simulink model "volo_agcdc_pipelined"  (R2012b)
settings: Solver=ode45  StartTime=0.0  StopTime=1000  RelTol=1e-3
PreLoadFcn:
  | volo_agcdc_init
InitFcn:
  | volo_agcdc_init
StartFcn:
  | volo_agcdc_init
values from neighbouring files (symbols this model uses):
  agc_idleState = 0    [volo_agcdc_init.m]
  agc_numAddrBits = agc_numOutputs + agc_numStateBits    [volo_agcdc_init.m]
  regDCRemoval_AvgLength = 64    [volo_agcdc_init.m]
  regSatDet_NumSamples = 16    [volo_agcdc_init.m]
undefined symbols (not defined in the file or in its folder): gcbh, xlBlockLoadCallback, xlGetNormalizedPeriod
libraries: xbsIndex_r4 x681, xbsEDKLib_r4 x1
(part 4 of 7)

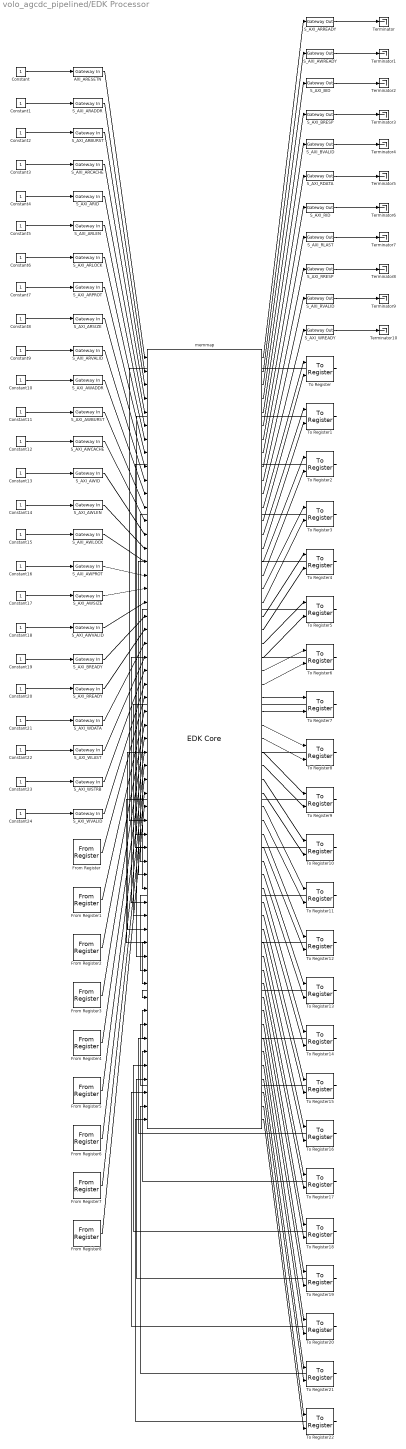
== system volo_agcdc_pipelined/EDK Processor ==
  AXI_ARESETN : xbsIndex_r4/Gateway In  gui_display_data_type=Fixed-point  arith_type=Boolean  n_bits=16  bin_pt=14  preci_type=Single  exp_width=8  frac_width=24  quantization="Round  (unbiased: +/- Inf)"  overflow=Saturate  period=xlGetNormalizedPeriod()  dbl_ovrd=off  timing_constraint=None  locs_specified=off  LOCs={}  UseAsADC=off  ADCChannel='1'  inherit_from_input=off  hdl_port=on  block_type=gatewayin
  Constant{,1..24} (25 alike) : Constant
  From Register : xbsIndex_r4/From Register  shared_memory_name='regSatDet_SaturationDetected'  init=0  period=xlGetNormalizedPeriod()  ownership=Owned and initialized elsewhere  gui_display_data_type=Fixed-point  arith_type=Unsigned  n_bits=1  bin_pt=0  preci_type=Single  dbl_ovrd=off  block_type=fromreg
      settings: AttributesFormatString=<< %<shared_memory_name> >>  infoedit="Register block that reads data to a shared memory register.  Delay of one sample period."
  From Register1 : xbsIndex_r4/From Register  shared_memory_name='regWSD_RXGAIN_READ'  init=0  period=xlGetNormalizedPeriod()  ownership=Owned and initialized elsewhere  gui_display_data_type=Fixed-point  arith_type="Signed  (2's comp)"  n_bits=9  bin_pt=0  preci_type=Single  dbl_ovrd=off  block_type=fromreg
      settings: AttributesFormatString=<< %<shared_memory_name> >>  infoedit="Register block that reads data to a shared memory register.  Delay of one sample period."
  From Register2 : xbsIndex_r4/From Register  shared_memory_name='regWSD_RSSI'  init=0  period=xlGetNormalizedPeriod()  ownership=Owned and initialized elsewhere  gui_display_data_type=Fixed-point  arith_type="Signed  (2's comp)"  n_bits=10  bin_pt=0  preci_type=Single  dbl_ovrd=off  block_type=fromreg
      settings: AttributesFormatString=<< %<shared_memory_name> >>  infoedit="Register block that reads data to a shared memory register.  Delay of one sample period."
  From Register3 : xbsIndex_r4/From Register  shared_memory_name='regWSD_meanPower'  init=0  period=xlGetNormalizedPeriod()  ownership=Owned and initialized elsewhere  gui_display_data_type=Fixed-point  arith_type="Signed  (2's comp)"  n_bits=9  bin_pt=0  preci_type=Single  dbl_ovrd=off  block_type=fromreg
      settings: AttributesFormatString=<< %<shared_memory_name> >>  infoedit="Register block that reads data to a shared memory register.  Delay of one sample period."
  From Register4 : xbsIndex_r4/From Register  shared_memory_name='regWSD_MeanDC_Q'  init=0  period=xlGetNormalizedPeriod()  ownership=Owned and initialized elsewhere  gui_display_data_type=Fixed-point  arith_type="Signed  (2's comp)"  n_bits=12  bin_pt=11  preci_type=Single  dbl_ovrd=off  block_type=fromreg
      settings: AttributesFormatString=<< %<shared_memory_name> >>  infoedit="Register block that reads data to a shared memory register.  Delay of one sample period."
  From Register5 : xbsIndex_r4/From Register  shared_memory_name='regWSD_MeanDC_I'  init=0  period=xlGetNormalizedPeriod()  ownership=Owned and initialized elsewhere  gui_display_data_type=Fixed-point  arith_type="Signed  (2's comp)"  n_bits=12  bin_pt=11  preci_type=Single  dbl_ovrd=off  block_type=fromreg
      settings: AttributesFormatString=<< %<shared_memory_name> >>  infoedit="Register block that reads data to a shared memory register.  Delay of one sample period."
  From Register6 : xbsIndex_r4/From Register  shared_memory_name='regWSD_RxLNAGain'  init=0  period=xlGetNormalizedPeriod()  ownership=Owned and initialized elsewhere  gui_display_data_type=Fixed-point  arith_type=Unsigned  n_bits=8  bin_pt=0  preci_type=Single  dbl_ovrd=off  block_type=fromreg
      settings: AttributesFormatString=<< %<shared_memory_name> >>  infoedit="Register block that reads data to a shared memory register.  Delay of one sample period."
  From Register7 : xbsIndex_r4/From Register  shared_memory_name='regWSD_RxVGA1Gain'  init=0  period=xlGetNormalizedPeriod()  ownership=Owned and initialized elsewhere  gui_display_data_type=Fixed-point  arith_type=Unsigned  n_bits=8  bin_pt=0  preci_type=Single  dbl_ovrd=off  block_type=fromreg
      settings: AttributesFormatString=<< %<shared_memory_name> >>  infoedit="Register block that reads data to a shared memory register.  Delay of one sample period."
  From Register8 : xbsIndex_r4/From Register  shared_memory_name='regWSD_RxVGA2Gain'  init=0  period=xlGetNormalizedPeriod()  ownership=Owned and initialized elsewhere  gui_display_data_type=Fixed-point  arith_type=Unsigned  n_bits=8  bin_pt=0  preci_type=Single  dbl_ovrd=off  block_type=fromreg
      settings: AttributesFormatString=<< %<shared_memory_name> >>  infoedit="Register block that reads data to a shared memory register.  Delay of one sample period."
  S_AXI_ARADDR : xbsIndex_r4/Gateway In  gui_display_data_type=Fixed-point  arith_type=Unsigned  n_bits=32  bin_pt=0  preci_type=Single  exp_width=8  frac_width=24  quantization="Round  (unbiased: +/- Inf)"  overflow=Saturate  period=xlGetNormalizedPeriod()  dbl_ovrd=off  timing_constraint=None  locs_specified=off  LOCs={}  UseAsADC=off  ADCChannel='1'  inherit_from_input=off  hdl_port=on  block_type=gatewayin
  S_AXI_ARBURST : xbsIndex_r4/Gateway In  gui_display_data_type=Fixed-point  arith_type=Unsigned  n_bits=2  bin_pt=0  preci_type=Single  exp_width=8  frac_width=24  quantization="Round  (unbiased: +/- Inf)"  overflow=Saturate  period=xlGetNormalizedPeriod()  dbl_ovrd=off  timing_constraint=None  locs_specified=off  LOCs={}  UseAsADC=off  ADCChannel='1'  inherit_from_input=off  hdl_port=on  block_type=gatewayin
  S_AXI_ARCACHE : xbsIndex_r4/Gateway In  gui_display_data_type=Fixed-point  arith_type=Unsigned  n_bits=4  bin_pt=0  preci_type=Single  exp_width=8  frac_width=24  quantization="Round  (unbiased: +/- Inf)"  overflow=Saturate  period=xlGetNormalizedPeriod()  dbl_ovrd=off  timing_constraint=None  locs_specified=off  LOCs={}  UseAsADC=off  ADCChannel='1'  inherit_from_input=off  hdl_port=on  block_type=gatewayin
  S_AXI_ARID : xbsIndex_r4/Gateway In  gui_display_data_type=Fixed-point  arith_type=Unsigned  n_bits=8  bin_pt=0  preci_type=Single  exp_width=8  frac_width=24  quantization="Round  (unbiased: +/- Inf)"  overflow=Saturate  period=xlGetNormalizedPeriod()  dbl_ovrd=off  timing_constraint=None  locs_specified=off  LOCs={}  UseAsADC=off  ADCChannel='1'  inherit_from_input=off  hdl_port=on  block_type=gatewayin
  S_AXI_ARLEN : xbsIndex_r4/Gateway In  gui_display_data_type=Fixed-point  arith_type=Unsigned  n_bits=8  bin_pt=0  preci_type=Single  exp_width=8  frac_width=24  quantization="Round  (unbiased: +/- Inf)"  overflow=Saturate  period=xlGetNormalizedPeriod()  dbl_ovrd=off  timing_constraint=None  locs_specified=off  LOCs={}  UseAsADC=off  ADCChannel='1'  inherit_from_input=off  hdl_port=on  block_type=gatewayin
  S_AXI_ARLOCK : xbsIndex_r4/Gateway In  gui_display_data_type=Fixed-point  arith_type=Unsigned  n_bits=2  bin_pt=0  preci_type=Single  exp_width=8  frac_width=24  quantization="Round  (unbiased: +/- Inf)"  overflow=Saturate  period=xlGetNormalizedPeriod()  dbl_ovrd=off  timing_constraint=None  locs_specified=off  LOCs={}  UseAsADC=off  ADCChannel='1'  inherit_from_input=off  hdl_port=on  block_type=gatewayin
  S_AXI_ARPROT : xbsIndex_r4/Gateway In  gui_display_data_type=Fixed-point  arith_type=Unsigned  n_bits=3  bin_pt=0  preci_type=Single  exp_width=8  frac_width=24  quantization="Round  (unbiased: +/- Inf)"  overflow=Saturate  period=xlGetNormalizedPeriod()  dbl_ovrd=off  timing_constraint=None  locs_specified=off  LOCs={}  UseAsADC=off  ADCChannel='1'  inherit_from_input=off  hdl_port=on  block_type=gatewayin
  S_AXI_ARREADY : xbsIndex_r4/Gateway Out  inherit_from_input=off  hdl_port=on  timing_constraint=None  locs_specified=off  LOCs={}  UseAsDAC=off  DACChannel='1'  block_type=gatewayout
  S_AXI_ARSIZE : xbsIndex_r4/Gateway In  gui_display_data_type=Fixed-point  arith_type=Unsigned  n_bits=3  bin_pt=0  preci_type=Single  exp_width=8  frac_width=24  quantization="Round  (unbiased: +/- Inf)"  overflow=Saturate  period=xlGetNormalizedPeriod()  dbl_ovrd=off  timing_constraint=None  locs_specified=off  LOCs={}  UseAsADC=off  ADCChannel='1'  inherit_from_input=off  hdl_port=on  block_type=gatewayin
  S_AXI_ARVALID : xbsIndex_r4/Gateway In  gui_display_data_type=Fixed-point  arith_type=Boolean  n_bits=16  bin_pt=14  preci_type=Single  exp_width=8  frac_width=24  quantization="Round  (unbiased: +/- Inf)"  overflow=Saturate  period=xlGetNormalizedPeriod()  dbl_ovrd=off  timing_constraint=None  locs_specified=off  LOCs={}  UseAsADC=off  ADCChannel='1'  inherit_from_input=off  hdl_port=on  block_type=gatewayin
  S_AXI_AWADDR : xbsIndex_r4/Gateway In  gui_display_data_type=Fixed-point  arith_type=Unsigned  n_bits=32  bin_pt=0  preci_type=Single  exp_width=8  frac_width=24  quantization="Round  (unbiased: +/- Inf)"  overflow=Saturate  period=xlGetNormalizedPeriod()  dbl_ovrd=off  timing_constraint=None  locs_specified=off  LOCs={}  UseAsADC=off  ADCChannel='1'  inherit_from_input=off  hdl_port=on  block_type=gatewayin
  S_AXI_AWBURST : xbsIndex_r4/Gateway In  gui_display_data_type=Fixed-point  arith_type=Unsigned  n_bits=2  bin_pt=0  preci_type=Single  exp_width=8  frac_width=24  quantization="Round  (unbiased: +/- Inf)"  overflow=Saturate  period=xlGetNormalizedPeriod()  dbl_ovrd=off  timing_constraint=None  locs_specified=off  LOCs={}  UseAsADC=off  ADCChannel='1'  inherit_from_input=off  hdl_port=on  block_type=gatewayin
  S_AXI_AWCACHE : xbsIndex_r4/Gateway In  gui_display_data_type=Fixed-point  arith_type=Unsigned  n_bits=4  bin_pt=0  preci_type=Single  exp_width=8  frac_width=24  quantization="Round  (unbiased: +/- Inf)"  overflow=Saturate  period=xlGetNormalizedPeriod()  dbl_ovrd=off  timing_constraint=None  locs_specified=off  LOCs={}  UseAsADC=off  ADCChannel='1'  inherit_from_input=off  hdl_port=on  block_type=gatewayin
  S_AXI_AWID : xbsIndex_r4/Gateway In  gui_display_data_type=Fixed-point  arith_type=Unsigned  n_bits=8  bin_pt=0  preci_type=Single  exp_width=8  frac_width=24  quantization="Round  (unbiased: +/- Inf)"  overflow=Saturate  period=xlGetNormalizedPeriod()  dbl_ovrd=off  timing_constraint=None  locs_specified=off  LOCs={}  UseAsADC=off  ADCChannel='1'  inherit_from_input=off  hdl_port=on  block_type=gatewayin
  S_AXI_AWLEN : xbsIndex_r4/Gateway In  gui_display_data_type=Fixed-point  arith_type=Unsigned  n_bits=8  bin_pt=0  preci_type=Single  exp_width=8  frac_width=24  quantization="Round  (unbiased: +/- Inf)"  overflow=Saturate  period=xlGetNormalizedPeriod()  dbl_ovrd=off  timing_constraint=None  locs_specified=off  LOCs={}  UseAsADC=off  ADCChannel='1'  inherit_from_input=off  hdl_port=on  block_type=gatewayin
  S_AXI_AWLOCK : xbsIndex_r4/Gateway In  gui_display_data_type=Fixed-point  arith_type=Unsigned  n_bits=2  bin_pt=0  preci_type=Single  exp_width=8  frac_width=24  quantization="Round  (unbiased: +/- Inf)"  overflow=Saturate  period=xlGetNormalizedPeriod()  dbl_ovrd=off  timing_constraint=None  locs_specified=off  LOCs={}  UseAsADC=off  ADCChannel='1'  inherit_from_input=off  hdl_port=on  block_type=gatewayin
  S_AXI_AWPROT : xbsIndex_r4/Gateway In  gui_display_data_type=Fixed-point  arith_type=Unsigned  n_bits=3  bin_pt=0  preci_type=Single  exp_width=8  frac_width=24  quantization="Round  (unbiased: +/- Inf)"  overflow=Saturate  period=xlGetNormalizedPeriod()  dbl_ovrd=off  timing_constraint=None  locs_specified=off  LOCs={}  UseAsADC=off  ADCChannel='1'  inherit_from_input=off  hdl_port=on  block_type=gatewayin
  S_AXI_AWREADY : xbsIndex_r4/Gateway Out  inherit_from_input=off  hdl_port=on  timing_constraint=None  locs_specified=off  LOCs={}  UseAsDAC=off  DACChannel='1'  block_type=gatewayout
  S_AXI_AWSIZE : xbsIndex_r4/Gateway In  gui_display_data_type=Fixed-point  arith_type=Unsigned  n_bits=3  bin_pt=0  preci_type=Single  exp_width=8  frac_width=24  quantization="Round  (unbiased: +/- Inf)"  overflow=Saturate  period=xlGetNormalizedPeriod()  dbl_ovrd=off  timing_constraint=None  locs_specified=off  LOCs={}  UseAsADC=off  ADCChannel='1'  inherit_from_input=off  hdl_port=on  block_type=gatewayin
  S_AXI_AWVALID : xbsIndex_r4/Gateway In  gui_display_data_type=Fixed-point  arith_type=Boolean  n_bits=16  bin_pt=14  preci_type=Single  exp_width=8  frac_width=24  quantization="Round  (unbiased: +/- Inf)"  overflow=Saturate  period=xlGetNormalizedPeriod()  dbl_ovrd=off  timing_constraint=None  locs_specified=off  LOCs={}  UseAsADC=off  ADCChannel='1'  inherit_from_input=off  hdl_port=on  block_type=gatewayin
  S_AXI_BID : xbsIndex_r4/Gateway Out  inherit_from_input=off  hdl_port=on  timing_constraint=None  locs_specified=off  LOCs={}  UseAsDAC=off  DACChannel='1'  block_type=gatewayout
  S_AXI_BREADY : xbsIndex_r4/Gateway In  gui_display_data_type=Fixed-point  arith_type=Boolean  n_bits=16  bin_pt=14  preci_type=Single  exp_width=8  frac_width=24  quantization="Round  (unbiased: +/- Inf)"  overflow=Saturate  period=xlGetNormalizedPeriod()  dbl_ovrd=off  timing_constraint=None  locs_specified=off  LOCs={}  UseAsADC=off  ADCChannel='1'  inherit_from_input=off  hdl_port=on  block_type=gatewayin
  S_AXI_BRESP : xbsIndex_r4/Gateway Out  inherit_from_input=off  hdl_port=on  timing_constraint=None  locs_specified=off  LOCs={}  UseAsDAC=off  DACChannel='1'  block_type=gatewayout
  S_AXI_BVALID : xbsIndex_r4/Gateway Out  inherit_from_input=off  hdl_port=on  timing_constraint=None  locs_specified=off  LOCs={}  UseAsDAC=off  DACChannel='1'  block_type=gatewayout
  S_AXI_RDATA : xbsIndex_r4/Gateway Out  inherit_from_input=off  hdl_port=on  timing_constraint=None  locs_specified=off  LOCs={}  UseAsDAC=off  DACChannel='1'  block_type=gatewayout
  S_AXI_RID : xbsIndex_r4/Gateway Out  inherit_from_input=off  hdl_port=on  timing_constraint=None  locs_specified=off  LOCs={}  UseAsDAC=off  DACChannel='1'  block_type=gatewayout
  S_AXI_RLAST : xbsIndex_r4/Gateway Out  inherit_from_input=off  hdl_port=on  timing_constraint=None  locs_specified=off  LOCs={}  UseAsDAC=off  DACChannel='1'  block_type=gatewayout
  S_AXI_RREADY : xbsIndex_r4/Gateway In  gui_display_data_type=Fixed-point  arith_type=Boolean  n_bits=16  bin_pt=14  preci_type=Single  exp_width=8  frac_width=24  quantization="Round  (unbiased: +/- Inf)"  overflow=Saturate  period=xlGetNormalizedPeriod()  dbl_ovrd=off  timing_constraint=None  locs_specified=off  LOCs={}  UseAsADC=off  ADCChannel='1'  inherit_from_input=off  hdl_port=on  block_type=gatewayin
  S_AXI_RRESP : xbsIndex_r4/Gateway Out  inherit_from_input=off  hdl_port=on  timing_constraint=None  locs_specified=off  LOCs={}  UseAsDAC=off  DACChannel='1'  block_type=gatewayout
  S_AXI_RVALID : xbsIndex_r4/Gateway Out  inherit_from_input=off  hdl_port=on  timing_constraint=None  locs_specified=off  LOCs={}  UseAsDAC=off  DACChannel='1'  block_type=gatewayout
  S_AXI_WDATA : xbsIndex_r4/Gateway In  gui_display_data_type=Fixed-point  arith_type=Unsigned  n_bits=32  bin_pt=0  preci_type=Single  exp_width=8  frac_width=24  quantization="Round  (unbiased: +/- Inf)"  overflow=Saturate  period=xlGetNormalizedPeriod()  dbl_ovrd=off  timing_constraint=None  locs_specified=off  LOCs={}  UseAsADC=off  ADCChannel='1'  inherit_from_input=off  hdl_port=on  block_type=gatewayin
  S_AXI_WLAST : xbsIndex_r4/Gateway In  gui_display_data_type=Fixed-point  arith_type=Boolean  n_bits=16  bin_pt=14  preci_type=Single  exp_width=8  frac_width=24  quantization="Round  (unbiased: +/- Inf)"  overflow=Saturate  period=xlGetNormalizedPeriod()  dbl_ovrd=off  timing_constraint=None  locs_specified=off  LOCs={}  UseAsADC=off  ADCChannel='1'  inherit_from_input=off  hdl_port=on  block_type=gatewayin
  S_AXI_WREADY : xbsIndex_r4/Gateway Out  inherit_from_input=off  hdl_port=on  timing_constraint=None  locs_specified=off  LOCs={}  UseAsDAC=off  DACChannel='1'  block_type=gatewayout
  S_AXI_WSTRB : xbsIndex_r4/Gateway In  gui_display_data_type=Fixed-point  arith_type=Unsigned  n_bits=4  bin_pt=0  preci_type=Single  exp_width=8  frac_width=24  quantization="Round  (unbiased: +/- Inf)"  overflow=Saturate  period=xlGetNormalizedPeriod()  dbl_ovrd=off  timing_constraint=None  locs_specified=off  LOCs={}  UseAsADC=off  ADCChannel='1'  inherit_from_input=off  hdl_port=on  block_type=gatewayin
  S_AXI_WVALID : xbsIndex_r4/Gateway In  gui_display_data_type=Fixed-point  arith_type=Boolean  n_bits=16  bin_pt=14  preci_type=Single  exp_width=8  frac_width=24  quantization="Round  (unbiased: +/- Inf)"  overflow=Saturate  period=xlGetNormalizedPeriod()  dbl_ovrd=off  timing_constraint=None  locs_specified=off  LOCs={}  UseAsADC=off  ADCChannel='1'  inherit_from_input=off  hdl_port=on  block_type=gatewayin
  Terminator{,1..10} (11 alike) : Terminator
  To Register : xbsIndex_r4/To Register  shared_memory_name='regAGC_DefaultGainSettings'  init=0  ownership=Owned and initialized elsewhere  explicit_data_type=on  gui_display_data_type=Fixed-point  arith_type=Unsigned  n_bits=32  bin_pt=0  preci_type=Single  dbl_ovrd=off  block_type=toreg
      settings: AttributesFormatString=<< %<shared_memory_name> >>  infoedit="Register block that writes data to a shared memory register.  Delay of one sample period."
  To Register1 : xbsIndex_r4/To Register  shared_memory_name='regSPICtrl_SPIWriteDelay'  init=0  ownership=Owned and initialized elsewhere  explicit_data_type=on  gui_display_data_type=Fixed-point  arith_type=Unsigned  n_bits=8  bin_pt=0  preci_type=Single  dbl_ovrd=off  block_type=toreg
      settings: AttributesFormatString=<< %<shared_memory_name> >>  infoedit="Register block that writes data to a shared memory register.  Delay of one sample period."
  To Register10 : xbsIndex_r4/To Register  shared_memory_name='regAGC_WSDAGCCtrl'  init=0  ownership=Owned and initialized elsewhere  explicit_data_type=on  gui_display_data_type=Fixed-point  arith_type=Unsigned  n_bits=32  bin_pt=0  preci_type=Single  dbl_ovrd=off  block_type=toreg
      settings: AttributesFormatString=<< %<shared_memory_name> >>  infoedit="Register block that writes data to a shared memory register.  Delay of one sample period."
  To Register11 : xbsIndex_r4/To Register  shared_memory_name='regAGC_AutoCorr_RatioThresh'  init=0  ownership=Owned and initialized elsewhere  explicit_data_type=on  gui_display_data_type=Fixed-point  arith_type=Unsigned  n_bits=8  bin_pt=8  preci_type=Single  dbl_ovrd=off  block_type=toreg
      settings: AttributesFormatString=<< %<shared_memory_name> >>  infoedit="Register block that writes data to a shared memory register.  Delay of one sample period."
  To Register12 : xbsIndex_r4/To Register  shared_memory_name='regAGC_ManualRxVGA1_Gain'  init=0  ownership=Owned and initialized elsewhere  explicit_data_type=on  gui_display_data_type=Fixed-point  arith_type=Unsigned  n_bits=8  bin_pt=0  preci_type=Single  dbl_ovrd=off  block_type=toreg
      settings: AttributesFormatString=<< %<shared_memory_name> >>  infoedit="Register block that writes data to a shared memory register.  Delay of one sample period."
  To Register13 : xbsIndex_r4/To Register  shared_memory_name='regAGC_ManualRxLNA_Gain'  init=0  ownership=Owned and initialized elsewhere  explicit_data_type=on  gui_display_data_type=Fixed-point  arith_type=Unsigned  n_bits=8  bin_pt=0  preci_type=Single  dbl_ovrd=off  block_type=toreg
      settings: AttributesFormatString=<< %<shared_memory_name> >>  infoedit="Register block that writes data to a shared memory register.  Delay of one sample period."
  To Register14 : xbsIndex_r4/To Register  shared_memory_name='regAGC_ManualRxVGA2_Gain'  init=0  ownership=Owned and initialized elsewhere  explicit_data_type=on  gui_display_data_type=Fixed-point  arith_type=Unsigned  n_bits=8  bin_pt=0  preci_type=Single  dbl_ovrd=off  block_type=toreg
      settings: AttributesFormatString=<< %<shared_memory_name> >>  infoedit="Register block that writes data to a shared memory register.  Delay of one sample period."
  To Register15 : xbsIndex_r4/To Register  shared_memory_name='regAGC_AutoCorr_LagTime'  init=0  ownership=Owned and initialized elsewhere  explicit_data_type=on  gui_display_data_type=Fixed-point  arith_type=Unsigned  n_bits=12  bin_pt=0  preci_type=Single  dbl_ovrd=off  block_type=toreg
      settings: AttributesFormatString=<< %<shared_memory_name> >>  infoedit="Register block that writes data to a shared memory register.  Delay of one sample period."
  To Register16 : xbsIndex_r4/To Register  shared_memory_name='regAGC_pktDetPwr_absoluteThreshold_dBm'  init=0  ownership=Owned and initialized elsewhere  explicit_data_type=on  gui_display_data_type=Fixed-point  arith_type="Signed  (2's comp)"  n_bits=9  bin_pt=0  preci_type=Single  dbl_ovrd=off  block_type=toreg
      settings: AttributesFormatString=<< %<shared_memory_name> >>  infoedit="Register block that writes data to a shared memory register.  Delay of one sample period."
  To Register17 : xbsIndex_r4/To Register  shared_memory_name='regAGC_pktDetPwr_detectLag'  init=0  ownership=Owned and initialized elsewhere  explicit_data_type=on  gui_display_data_type=Fixed-point  arith_type=Unsigned  n_bits=6  bin_pt=0  preci_type=Single  dbl_ovrd=off  block_type=toreg
      settings: AttributesFormatString=<< %<shared_memory_name> >>  infoedit="Register block that writes data to a shared memory register.  Delay of one sample period."
  To Register18 : xbsIndex_r4/To Register  shared_memory_name='regAGC_NumFineGainSteps'  init=0  ownership=Owned and initialized elsewhere  explicit_data_type=on  gui_display_data_type=Fixed-point  arith_type=Unsigned  n_bits=4  bin_pt=0  preci_type=Single  dbl_ovrd=off  block_type=toreg
      settings: AttributesFormatString=<< %<shared_memory_name> >>  infoedit="Register block that writes data to a shared memory register.  Delay of one sample period."
  To Register19 : xbsIndex_r4/To Register  shared_memory_name='regAGC_WSD_CCAThreshold_dBm'  init=0  ownership=Owned and initialized elsewhere  explicit_data_type=on  gui_display_data_type=Fixed-point  arith_type=Unsigned  n_bits=10  bin_pt=0  preci_type=Single  dbl_ovrd=off  block_type=toreg
      settings: AttributesFormatString=<< %<shared_memory_name> >>  infoedit="Register block that writes data to a shared memory register.  Delay of one sample period."
  To Register2 : xbsIndex_r4/To Register  shared_memory_name='regPwrMeas_AvgLength'  init=0  ownership=Owned and initialized elsewhere  explicit_data_type=on  gui_display_data_type=Fixed-point  arith_type=Unsigned  n_bits=7  bin_pt=0  preci_type=Single  dbl_ovrd=off  block_type=toreg
      settings: AttributesFormatString=<< %<shared_memory_name> >>  infoedit="Register block that writes data to a shared memory register.  Delay of one sample period."
  To Register20 : xbsIndex_r4/To Register  shared_memory_name='regAGC_LongCorr_Threshold'  init=0  ownership=Owned and initialized elsewhere  explicit_data_type=on  gui_display_data_type=Fixed-point  arith_type=Unsigned  n_bits=32  bin_pt=0  preci_type=Single  dbl_ovrd=off  block_type=toreg
      settings: AttributesFormatString=<< %<shared_memory_name> >>  infoedit="Register block that writes data to a shared memory register.  Delay of one sample period."
  To Register21 : xbsIndex_r4/To Register  shared_memory_name='regAGC_pktDetPwr_deltaThreshold_dBm'  init=0  ownership=Owned and initialized elsewhere  explicit_data_type=on  gui_display_data_type=Fixed-point  arith_type="Signed  (2's comp)"  n_bits=9  bin_pt=0  preci_type=Single  dbl_ovrd=off  block_type=toreg
      settings: AttributesFormatString=<< %<shared_memory_name> >>  infoedit="Register block that writes data to a shared memory register.  Delay of one sample period."
  To Register22 : xbsIndex_r4/To Register  shared_memory_name='regAGC_SPITIMINGFUDGE'  init=0  ownership=Owned and initialized elsewhere  explicit_data_type=on  gui_display_data_type=Fixed-point  arith_type=Unsigned  n_bits=12  bin_pt=0  preci_type=Single  dbl_ovrd=off  block_type=toreg
      settings: AttributesFormatString=<< %<shared_memory_name> >>  infoedit="Register block that writes data to a shared memory register.  Delay of one sample period."
  To Register3 : xbsIndex_r4/To Register  shared_memory_name='regSatDet_SaturationMaxCount'  init=0  ownership=Owned and initialized elsewhere  explicit_data_type=on  gui_display_data_type=Fixed-point  arith_type=Unsigned  n_bits=6  bin_pt=0  preci_type=Single  dbl_ovrd=off  block_type=toreg
      settings: AttributesFormatString=<< %<shared_memory_name> >>  infoedit="Register block that writes data to a shared memory register.  Delay of one sample period."
  To Register4 : xbsIndex_r4/To Register  shared_memory_name='regSatDet_NumSamples'  init=0  ownership=Owned and initialized elsewhere  explicit_data_type=on  gui_display_data_type=Fixed-point  arith_type=Unsigned  n_bits=5  bin_pt=0  preci_type=Single  dbl_ovrd=off  block_type=toreg
      settings: AttributesFormatString=<< %<shared_memory_name> >>  infoedit="Register block that writes data to a shared memory register.  Delay of one sample period."
  To Register5 : xbsIndex_r4/To Register  shared_memory_name='regSatDet_SaturationThreshold'  init=0  ownership=Owned and initialized elsewhere  explicit_data_type=on  gui_display_data_type=Fixed-point  arith_type="Signed  (2's comp)"  n_bits=14  bin_pt=13  preci_type=Single  dbl_ovrd=off  block_type=toreg
      settings: AttributesFormatString=<< %<shared_memory_name> >>  infoedit="Register block that writes data to a shared memory register.  Delay of one sample period."
  To Register6 : xbsIndex_r4/To Register  shared_memory_name='regAGC_ExtPktDet_DelayCount'  init=0  ownership=Owned and initialized elsewhere  explicit_data_type=on  gui_display_data_type=Fixed-point  arith_type=Unsigned  n_bits=32  bin_pt=0  preci_type=Single  dbl_ovrd=off  block_type=toreg
      settings: AttributesFormatString=<< %<shared_memory_name> >>  infoedit="Register block that writes data to a shared memory register.  Delay of one sample period."
  To Register7 : xbsIndex_r4/To Register  shared_memory_name='regAGC_targetRxInputPwr'  init=0  ownership=Owned and initialized elsewhere  explicit_data_type=on  gui_display_data_type=Fixed-point  arith_type="Signed  (2's comp)"  n_bits=9  bin_pt=0  preci_type=Single  dbl_ovrd=off  block_type=toreg
      settings: AttributesFormatString=<< %<shared_memory_name> >>  infoedit="Register block that writes data to a shared memory register.  Delay of one sample period."
  To Register8 : xbsIndex_r4/To Register  shared_memory_name='regAGC_AutoCorr_MinPower'  init=0  ownership=Owned and initialized elsewhere  explicit_data_type=on  gui_display_data_type=Fixed-point  arith_type=Unsigned  n_bits=16  bin_pt=8  preci_type=Single  dbl_ovrd=off  block_type=toreg
      settings: AttributesFormatString=<< %<shared_memory_name> >>  infoedit="Register block that writes data to a shared memory register.  Delay of one sample period."
  To Register9 : xbsIndex_r4/To Register  shared_memory_name='regAGC_AutoCorr_MinPktDuration'  init=0  ownership=Owned and initialized elsewhere  explicit_data_type=on  gui_display_data_type=Fixed-point  arith_type=Unsigned  n_bits=6  bin_pt=0  preci_type=Single  dbl_ovrd=off  block_type=toreg
      settings: AttributesFormatString=<< %<shared_memory_name> >>  infoedit="Register block that writes data to a shared memory register.  Delay of one sample period."
  memmap : xbsEDKLib_r4/EDK Core  sim_method=Inactive  xmp=xmp  blockname=blockname  dual_clock=dual_clock  procinfo=procinfo  bus_type=bus_type  memxtable=memxtable  memmap_hdlcontent=|  config={'inports'=>[{'arith_type'=>2.00000000000000000,'bin_pt'=>0.00000000000000000,'name'=>'AXI_ARESETN','width'=>0},{'arith_type'=>2.00000000000000000,'bin_pt'=>0.00000000000000000,'name'=>'S_AXI_ARADDR','width'=>32},{'arith_type'=>2.00000000000000000,'bin_pt'=>0.00000000000000000,'name'=>'S_AXI_ARBURST','width'=>2},{'arith_type'=>2.00000000000000000,'bin_pt'=>0.00000000000000000,'name'=>'S_AXI_ARCACHE','width'=>4},{'arith_type'=>2.00000000000000000,'bin_pt'=>0.00000000000000000,'name'=>'S_AXI_ARID','width'=>8},{'arith_type'=>2.00000000000000000,'bin_pt'=>0.00000000000000000,'name'=>'S_AXI_ARLEN','width'=>8},{'arith_type'=>2.00000000000000000,'bin_pt'=>0.00000000000000000,'name'=>'S_AXI_ARLOCK','width'=>2},{'arith_type'=>2.00000000000000000,'bin_pt'=>0.00000000000000000,'name'=>'S_AXI_ARPROT','width'=>3},{'arith_type'=>2.00000000000000000,'bin_pt'=>0.00000000000000000,'name'=>'S_AXI_ARSIZE','width'=>3},{'arith_type'=>2.00000000000000000,'bin_pt'=>0.00000000000000000,'name'=>'S_AXI_ARVALID','width'=>0},{'arith_type'=>2.00000000000000000,'bin_pt'=>0.00000000000000000,'name'=>'S_AXI_AWADDR','width'=>32},{'arith_type'=>2.00000000000000000,'bin_pt'=>0.00000000000000000,'name'=>'S_AXI_AWBURST','width'=>2},{'arith_type'=>2.00000000000000000,'bin_pt'=>0.00000000000000000,'name'=>'S_AXI_AWCACHE','width'=>4},{'arith_type'=>2.00000000000000000,'bin_pt'=>0.00000000000000000,'name'=>'S_AXI_AWID','width'=>8},{'arith_type'=>2.00000000000000000,'bin_pt'=>0.00000000000000000,'name'=>'S_AXI_AWLEN','width'=>8},{'arith_type'=>2.00000000000000000,'bin_pt'=>0.00000000000000000,'name'=>'S_AXI_AWLOCK','width'=>2},{'arith_type'=>2.00000000000000000,'bin_pt'=>0.00000000000000000,'name'=>'S_AXI_AWPROT','width'=>3},{'arith_type'=>2.00000000000000000,'bin_pt'=>0.00000000000000000,'name'=>'S_AXI_AWSIZE','width'=>3},{'arith_type'=>2.00000000000000000,'bin_pt'=>0.00000000000000000,'name'=>'S_AXI_AWVALID','width'=>0},{'arith_type'=>2.00000000000000000,'bin_pt'=>0.00000000000000000,'name'=>'S_AXI_BREADY','width'=>0},{'arith_type'=>2.00000000000000000,'bin_pt'=>0.00000000000000000,'name'=>'S_AXI_RREADY','width'=>0},{'arith_type'=>2.00000000000000000,'bin_pt'=>0.00000000000000000,'name'=>'S_AXI_WDATA','width'=>32},{'arith_type'=>2.00000000000000000,'bin_pt'=>0.00000000000000000,'name'=>'S_AXI_WLAST','width'=>0},{'arith_type'=>2.00000000000000000,'bin_pt'=>0.00000000000000000,'name'=>'S_AXI_WSTRB','width'=>4},{'arith_type'=>2.00000000000000000,'bin_pt'=>0.00000000000000000,'name'=>'S_AXI_WVALID','width'=>0},{'arith_type'=>2,'bin_pt'=>0,'name'=>'sm_regSatDet_SaturationDetected_dout','width'=>1},{'arith_type'=>1,'bin_pt'=>0,'name'=>'sm_regWSD_RXGAIN_READ_dout','width'=>9},{'arith_type'=>1,'bin_pt'=>0,'name'=>'sm_regWSD_RSSI_dout','width'=>10},{'arith_type'=>1,'bin_pt'=>0,'name'=>'sm_regWSD_meanPower_dout','width'=>9},{'arith_type'=>1,'bin_pt'=>11,'name'=>'sm_regWSD_MeanDC_Q_dout','width'=>12},{'arith_type'=>1,'bin_pt'=>11,'name'=>'sm_regWSD_MeanDC_I_dout','width'=>12},{'arith_type'=>2,'bin_pt'=>0,'name'=>'sm_regWSD_RxLNAGain_dout','width'=>8},{'arith_type'=>2,'bin_pt'=>0,'name'=>'sm_regWSD_RxVGA1Gain_dout','width'=>8},{'arith_type'=>2,'bin_pt'=>0,'name'=>'sm_regWSD_RxVGA2Gain_dout','width'=>8},{'arith_type'=>2,'bin_pt'=>0,'name'=>'sm_regAGC_DefaultGainSettings_dout','width'=>32},{'arith_type'=>2,'bin_pt'=>0,'name'=>'sm_regSPICtrl_SPIWriteDelay_dout','width'=>8},{'arith_type'=>2,'bin_pt'=>0,'name'=>'sm_regPwrMeas_AvgLength_dout','width'=>7},{'arith_type'=>2,'bin_pt'=>0,'name'=>'sm_regSatDet_SaturationMaxCount_dout','width'=>6},{'arith_type'=>2,'bin_pt'=>0,'name'=>'sm_regSatDet_NumSamples_dout','width'=>5},{'arith_type'=>1,'bin_pt'=>13,'name'=>'sm_regSatDet_SaturationThreshold_dout','width'=>14},{'arith_type'=>2,'bin_pt'=>0,'name'=>'sm_regAGC_ExtPktDet_DelayCount_dout','width'=>32},{'arith_type'=>1,'bin_pt'=>0,'name'=>'sm_regAGC_targetRxInputPwr_dout','width'=>9},{'arith_type'=>2,'bin_pt'=>8,'name'=>'sm_regAGC_AutoCorr_MinPower_dout','width'=>16},{'arith_type'=>2,'bin_pt'=>0,'name'=>'sm_regAGC_AutoCorr_MinPktDuration_dout','width'=>6},{'arith_type'=>2,'bin_pt'=>0,'name'=>'sm_regAGC_WSDAGCCtrl_dout','width'=>32},{'arith_type'=>2,'bin_pt'=>8,'name'=>'sm_regAGC_AutoCorr_RatioThresh_dout','width'=>8},{'arith_type'=>2,'bin_pt'=>0,'name'=>'sm_regAGC_ManualRxVGA1_Gain_dout','width'=>8},{'arith_type'=>2,'bin_pt'=>0,'name'=>'sm_regAGC_ManualRxLNA_Gain_dout','width'=>8},{'arith_type'=>2,'bin_pt'=>0,'name'=>'sm_regAGC_ManualRxVGA2_Gain_dout','width'=>8},{'arith_type'=>2,'bin_pt'=>0,'name'=>'sm_regAGC_AutoCorr_LagTime_dout','width'=>12},{'arith_type'=>1,'bin_pt'=>0,'name'=>'sm_regAGC_pktDetPwr_absoluteThreshold_dBm_dout','width'=>9},{'arith_type'=>2,'bin_pt'=>0,'name'=>'sm_regAGC_pktDetPwr_detectLag_dout','width'=>6},{'arith_type'=>2,'bin_pt'=>0,'name'=>'sm_regAGC_NumFineGainSteps_dout','width'=>4},{'arith_type'=>2,'bin_pt'=>0,'name'=>'sm_regAGC_WSD_CCAThreshold_dBm_dout','width'=>10},{'arith_type'=>2,'bin_pt'=>0,'name'=>'sm_regAGC_LongCorr_Threshold_dout','width'=>32},{'arith_type'=>1,'bin_pt'=>0,'name'=>'sm_regAGC_pktDetPwr_deltaThreshold_dBm_dout','width'=>9},{'arith_type'=>2,'bin_pt'=>0,'name'=>'sm_regAGC_SPITIMINGFUDGE_dout','width'=>12}],'outports'=>[{'arith_type'=>2.00000000000000000,'bin_pt'=>0.00000000000000000,'name'=>'S_AXI_ARREADY','width'=>0},{'arith_type'=>2.00000000000000000,'bin_pt'=>0.00000000000000000,'name'=>'S_AXI_AWREADY','width'=>0},{'arith_type'=>2.00000000000000000,'bin_pt'=>0.00000000000000000,'name'=>'S_AXI_BID','width'=>8},{'arith_type'=>2.00000000000000000,'bin_pt'=>0.00000000000000000,'name'=>'S_AXI_BRESP','width'=>2},{'arith_type'=>2.00000000000000000,'bin_pt'=>0.00000000000000000,'name'=>'S_AXI_BVALID','width'=>0},{'arith_type'=>2.00000000000000000,'bin_pt'=>0.00000000000000000,'name'=>'S_AXI_RDATA','width'=>32},{'arith_type'=>2.00000000000000000,'bin_pt'=>0.00000000000000000,'name'=>'S_AXI_RID','width'=>8},{'arith_type'=>2.00000000000000000,'bin_pt'=>0.00000000000000000,'name'=>'S_AXI_RLAST','width'=>0},{'arith_type'=>2.00000000000000000,'bin_pt'=>0.00000000000000000,'name'=>'S_AXI_RRESP','width'=>2},{'arith_type'=>2.00000000000000000,'bin_pt'=>0.00000000000000000,'name'=>'S_AXI_RVALID','width'=>0},{'arith_type'=>2.00000000000000000,'bin_pt'=>0.00000000000000000,'name'=>'S_AXI_WREADY','width'=>0},{'arith_type'=>2,'bin_pt'=>0,'name'=>'sm_regAGC_DefaultGainSettings_din','width'=>32},{'arith_type'=>2.00000000000000000,'bin_pt'=>0.00000000000000000,'name'=>'sm_regAGC_DefaultGainSettings_en','width'=>0.00000000000000000},{'arith_type'=>2,'bin_pt'=>0,'name'=>'sm_regSPICtrl_SPIWriteDelay_din','width'=>8},{'arith_type'=>2.00000000000000000,'bin_pt'=>0.00000000000000000,'name'=>'sm_regSPICtrl_SPIWriteDelay_en','width'=>0.00000000000000000},{'arith_type'=>2,'bin_pt'=>0,'name'=>'sm_regPwrMeas_AvgLength_din','width'=>7},{'arith_type'=>2.00000000000000000,'bin_pt'=>0.00000000000000000,'name'=>'sm_regPwrMeas_AvgLength_en','width'=>0.00000000000000000},{'arith_type'=>2,'bin_pt'=>0,'name'=>'sm_regSatDet_SaturationMaxCount_din','width'=>6},{'arith_type'=>2.00000000000000000,'bin_pt'=>0.00000000000000000,'name'=>'sm_regSatDet_SaturationMaxCount_en','width'=>0.00000000000000000},{'arith_type'=>2,'bin_pt'=>0,'name'=>'sm_regSatDet_NumSamples_din','width'=>5},{'arith_type'=>2.00000000000000000,'bin_pt'=>0.00000000000000000,'name'=>'sm_regSatDet_NumSamples_en','width'=>0.00000000000000000},{'arith_type'=>1,'bin_pt'=>13,'name'=>'sm_regSatDet_SaturationThreshold_din','width'=>14},{'arith_type'=>2.00000000000000000,'bin_pt'=>0.00000000000000000,'name'=>'sm_regSatDet_SaturationThreshold_en','width'=>0.00000000000000000},{'arith_type'=>2,'bin_pt'=>0,'name'=>'sm_regAGC_ExtPktDet_DelayCount_din','width'=>32},{'arith_type'=>2.00000000000000000,'bin_pt'=>0.00000000000000000,'name'=>'sm_regAGC_ExtPktDet_DelayCount_en','width'=>0.00000000000000000},{'arith_type'=>1,'bin_pt'=>0,'name'=>'sm_regAGC_targetRxInputPwr_din','width'=>9},{'arith_type'=>2.00000000000000000,'bin_pt'=>0.00000000000000000,'name'=>'sm_regAGC_targetRxInputPwr_en','width'=>0.00000000000000000},{'arith_type'=>2,'bin_pt'=>8,'name'=>'sm_regAGC_AutoCorr_MinPower_din','width'=>16},{'arith_type'=>2.00000000000000000,'bin_pt'=>0.00000000000000000,'name'=>'sm_regAGC_AutoCorr_MinPower_en','width'=>0.00000000000000000},{'arith_type'=>2,'bin_pt'=>0,'name'=>'sm_regAGC_AutoCorr_MinPktDuration_din','width'=>6},{'arith_type'=>2.00000000000000000,'bin_pt'=>0.00000000000000000,'name'=>'sm_regAGC_AutoCorr_MinPktDuration_en','width'=>0.00000000000000000},{'arith_type'=>2,'bin_pt'=>0,'name'=>'sm_regAGC_WSDAGCCtrl_din','width'=>32},{'arith_type'=>2.00000000000000000,'bin_pt'=>0.00000000000000000,'name'=>'sm_regAGC_WSDAGCCtrl_en','width'=>0.00000000000000000},{'arith_type'=>2,'bin_pt'=>8,'name'=>'sm_regAGC_AutoCorr_RatioThresh_din','width'=>8},{'arith_type'=>2.00000000000000000,'bin_pt'=>0.00000000000000000,'name'=>'sm_regAGC_AutoCorr_RatioThresh_en','width'=>0.00000000000000000},{'arith_type'=>2,'bin_pt'=>0,'name'=>'sm_regAGC_ManualRxVGA1_Gain_din','width'=>8},{'arith_type'=>2.00000000000000000,'bin_pt'=>0.00000000000000000,'name'=>'sm_regAGC_ManualRxVGA1_Gain_en','width'=>0.00000000000000000},{'arith_type'=>2,'bin_pt'=>0,'name'=>'sm_regAGC_ManualRxLNA_Gain_din','width'=>8},{'arith_type'=>2.00000000000000000,'bin_pt'=>0.00000000000000000,'name'=>'sm_regAGC_ManualRxLNA_Gain_en','width'=>0.00000000000000000},{'arith_type'=>2,'bin_pt'=>0,'name'=>'sm_regAGC_ManualRxVGA2_Gain_din','width'=>8},{'arith_type'=>2.00000000000000000,'bin_pt'=>0.00000000000000000,'name'=>'sm_regAGC_ManualRxVGA2_Gain_en','width'=>0.00000000000000000},{'arith_type'=>2,'bin_pt'=>0,'name'=>'sm_regAGC_AutoCorr_LagTime_din','width'=>12},{'arith_type'=>2.00000000000000000,'bin_pt'=>0.00000000000000000,'name'=>'sm_regAGC_AutoCorr_LagTime_en','width'=>0.00000000000000000},{'arith_type'=>1,'bin_pt'=>0,'name'=>'sm_regAGC_pktDetPwr_absoluteThreshold_dBm_din','width'=>9},{'arith_type'=>2.00000000000000000,'bin_pt'=>0.00000000000000000,'name'=>'sm_regAGC_pktDetPwr_absoluteThreshold_dBm_en','width'=>0.00000000000000000},{'arith_type'=>2,'bin_pt'=>0,'name'=>'sm_regAGC_pktDetPwr_detectLag_din','width'=>6},{'arith_type'=>2.00000000000000000,'bin_pt'=>0.00000000000000000,'name'=>'sm_regAGC_pktDetPwr_detectLag_en','width'=>0.00000000000000000},{'arith_type'=>2,'bin_pt'=>0,'name'=>'sm_regAGC_NumFineGainSteps_din','width'=>4},{'arith_type'=>2.00000000000000000,'bin_pt'=>0.00000000000000000,'name'=>'sm_regAGC_NumFineGainSteps_en','width'=>0.00000000000000000},{'arith_type'=>2,'bin_pt'=>0,'name'=>'sm_regAGC_WSD_CCAThreshold_dBm_din','width'=>10},{'arith_type'=>2.00000000000000000,'bin_pt'=>0.00000000000000000,'name'=>'sm_regAGC_WSD_CCAThreshold_dBm_en','width'=>0.00000000000000000},{'arith_type'=>2,'bin_pt'=>0,'name'=>'sm_regAGC_LongCorr_Threshold_din','width'=>32},{'arith_type'=>2.00000000000000000,'bin_pt'=>0.00000000000000000,'name'=>'sm_regAGC_LongCorr_Threshold_en','width'=>0.00000000000000000},{'arith_type'=>1,'bin_pt'=>0,'name'=>'sm_regAGC_pktDetPwr_deltaThreshold_dBm_din','width'=>9},{'arith_type'=>2.00000000000000000,'bin_pt'=>0.00000000000000000,'name'=>'sm_regAGC_pktDetPwr_deltaThreshold_dBm_en','width'=>0.00000000000000000},{'arith_type'=>2,'bin_pt'=>0,'name'=>'sm_regAGC_SPITIMINGFUDGE_din','width'=>12},{'arith_type'=>2.00000000000000000,'bin_pt'=>0.00000000000000000,'name'=>'sm_regAGC_SPITIMINGFUDGE_en','width'=>0.00000000000000000}]}  inheritDeviceType=inheritDeviceType  block_type=edkcore
      | library IEEE;
      | use IEEE.std_logic_1164.all;
      | use IEEE.numeric_std.all;
      | 
      | entity axi_sgiface is
      |     generic (
      |         -- AXI specific.
      |         -- TODO: need to figure out a way to pass these generics from outside
      |         C_S_AXI_SUPPORT_BURST   : integer := 0;
      |         -- TODO: fix the internal ID width to 8
      |         C_S_AXI_ID_WIDTH        : integer := 8;
      |         C_S_AXI_DATA_WIDTH      : integer := 32;
      |         C_S_AXI_ADDR_WIDTH      : integer := 32;
      |         C_S_AXI_TOTAL_ADDR_LEN  : integer := 12;
      |         C_S_AXI_LINEAR_ADDR_LEN : integer := 8;
      |         C_S_AXI_BANK_ADDR_LEN   : integer := 2;
      |         C_S_AXI_AWLEN_WIDTH     : integer := 8;
      |         C_S_AXI_ARLEN_WIDTH     : integer := 8
      |     );
      |     port (
      |         -- General.
      |         AXI_AClk      : in  std_logic;
      |         AXI_AResetN    : in  std_logic;
      |         -- not used
      |         AXI_Ce        : in  std_logic;
      |   
      |         -- AXI Port.
      |         S_AXI_AWADDR  : in  std_logic_vector(C_S_AXI_ADDR_WIDTH-1 downto 0);
      |         S_AXI_AWID    : in  std_logic_vector(C_S_AXI_ID_WIDTH-1 downto 0);
      |         S_AXI_AWLEN   : in  std_logic_vector(C_S_AXI_AWLEN_WIDTH-1 downto 0);
      |         S_AXI_AWSIZE  : in  std_logic_vector(2 downto 0);
      |         S_AXI_AWBURST : in  std_logic_vector(1 downto 0);
      |         S_AXI_AWLOCK  : in  std_logic_vector(1 downto 0);
      |         S_AXI_AWCACHE : in  std_logic_vector(3 downto 0);
      |         S_AXI_AWPROT  : in  std_logic_vector(2 downto 0);
      |         S_AXI_AWVALID : in  std_logic;
      |         S_AXI_AWREADY : out std_logic;
      |         
      |         S_AXI_WLAST   : in  std_logic;
      |         S_AXI_WDATA   : in  std_logic_vector(C_S_AXI_DATA_WIDTH-1 downto 0);
      |         S_AXI_WSTRB   : in  std_logic_vector((C_S_AXI_DATA_WIDTH/8)-1 downto 0);
      |         S_AXI_WVALID  : in  std_logic;
      |         S_AXI_WREADY  : out std_logic;
      |         
      |         S_AXI_BRESP   : out std_logic_vector(1 downto 0);
      |         S_AXI_BID     : out std_logic_vector(C_S_AXI_ID_WIDTH-1 downto 0);
      |         S_AXI_BVALID  : out std_logic;
      |         S_AXI_BREADY  : in  std_logic;
      |         
      |         S_AXI_ARADDR  : in  std_logic_vector(C_S_AXI_ADDR_WIDTH-1 downto 0);
      |         S_AXI_ARID    : in  std_logic_vector(C_S_AXI_ID_WIDTH-1 downto 0);
      |         S_AXI_ARLEN   : in  std_logic_vector(C_S_AXI_ARLEN_WIDTH-1 downto 0);
      |         S_AXI_ARSIZE  : in  std_logic_vector(2 downto 0);
      |         S_AXI_ARBURST : in  std_logic_vector(1 downto 0);
      |         S_AXI_ARLOCK  : in  std_logic_vector(1 downto 0);
      |         S_AXI_ARCACHE : in  std_logic_vector(3 downto 0);
      |         S_AXI_ARPROT  : in  std_logic_vector(2 downto 0);
      |         S_AXI_ARVALID : in  std_logic;
      |         S_AXI_ARREADY : out std_logic;
      |         
      |         -- 'From Register'
      |         -- 'regSatDet_SaturationDetected'
      |         sm_regSatDet_SaturationDetected_dout : in std_logic_vector(1-1 downto 0);
      |         -- 'regWSD_RXGAIN_READ'
      |         sm_regWSD_RXGAIN_READ_dout : in std_logic_vector(9-1 downto 0);
      |         -- 'regWSD_RSSI'
      |         sm_regWSD_RSSI_dout : in std_logic_vector(10-1 downto 0);
      |         -- 'regWSD_meanPower'
      |         sm_regWSD_meanPower_dout : in std_logic_vector(9-1 downto 0);
      |         -- 'regWSD_MeanDC_Q'
      |         sm_regWSD_MeanDC_Q_dout : in std_logic_vector(12-1 downto 0);
      |         -- 'regWSD_MeanDC_I'
      |         sm_regWSD_MeanDC_I_dout : in std_logic_vector(12-1 downto 0);
      |         -- 'regWSD_RxLNAGain'
      |         sm_regWSD_RxLNAGain_dout : in std_logic_vector(8-1 downto 0);
      |         -- 'regWSD_RxVGA1Gain'
      |         sm_regWSD_RxVGA1Gain_dout : in std_logic_vector(8-1 downto 0);
      |         -- 'regWSD_RxVGA2Gain'
      |         sm_regWSD_RxVGA2Gain_dout : in std_logic_vector(8-1 downto 0);
      |         -- 'To Register'
      |         -- 'regAGC_DefaultGainSettings'
      |         sm_regAGC_DefaultGainSettings_dout : in std_logic_vector(32-1 downto 0);
      |         sm_regAGC_DefaultGainSettings_din  : out std_logic_vector(32-1 downto 0);
      |         sm_regAGC_DefaultGainSettings_en   : out std_logic;
      |         -- 'regSPICtrl_SPIWriteDelay'
      |         sm_regSPICtrl_SPIWriteDelay_dout : in std_logic_vector(8-1 downto 0);
      |         sm_regSPICtrl_SPIWriteDelay_din  : out std_logic_vector(8-1 downto 0);
      |         sm_regSPICtrl_SPIWriteDelay_en   : out std_logic;
      |         -- 'regPwrMeas_AvgLength'
      |         sm_regPwrMeas_AvgLength_dout : in std_logic_vector(7-1 downto 0);
      |         sm_regPwrMeas_AvgLength_din  : out std_logic_vector(7-1 downto 0);
      |         sm_regPwrMeas_AvgLength_en   : out std_logic;
      |         -- 'regSatDet_SaturationMaxCount'
      |         sm_regSatDet_SaturationMaxCount_dout : in std_logic_vector(6-1 downto 0);
      |         sm_regSatDet_SaturationMaxCount_din  : out std_logic_vector(6-1 downto 0);
      |         sm_regSatDet_SaturationMaxCount_en   : out std_logic;
      |         -- 'regSatDet_NumSamples'
      |         sm_regSatDet_NumSamples_dout : in std_logic_vector(5-1 downto 0);
      |         sm_regSatDet_NumSamples_din  : out std_logic_vector(5-1 downto 0);
      |         sm_regSatDet_NumSamples_en   : out std_logic;
      |         -- 'regSatDet_SaturationThreshold'
      |         sm_regSatDet_SaturationThreshold_dout : in std_logic_vector(14-1 downto 0);
      |         sm_regSatDet_SaturationThreshold_din  : out std_logic_vector(14-1 downto 0);
      |         sm_regSatDet_SaturationThreshold_en   : out std_logic;
      |         -- 'regAGC_ExtPktDet_DelayCount'
      |         sm_regAGC_ExtPktDet_DelayCount_dout : in std_logic_vector(32-1 downto 0);
      |         sm_regAGC_ExtPktDet_DelayCount_din  : out std_logic_vector(32-1 downto 0);
      |         sm_regAGC_ExtPktDet_DelayCount_en   : out std_logic;
      |         -- 'regAGC_targetRxInputPwr'
      |         sm_regAGC_targetRxInputPwr_dout : in std_logic_vector(9-1 downto 0);
      |         sm_regAGC_targetRxInputPwr_din  : out std_logic_vector(9-1 downto 0);
      |         sm_regAGC_targetRxInputPwr_en   : out std_logic;
      |         -- 'regAGC_AutoCorr_MinPower'
      |         sm_regAGC_AutoCorr_MinPower_dout : in std_logic_vector(16-1 downto 0);
      |         sm_regAGC_AutoCorr_MinPower_din  : out std_logic_vector(16-1 downto 0);
      |         sm_regAGC_AutoCorr_MinPower_en   : out std_logic;
      |         -- 'regAGC_AutoCorr_MinPktDuration'
      |         sm_regAGC_AutoCorr_MinPktDuration_dout : in std_logic_vector(6-1 downto 0);
      |         sm_regAGC_AutoCorr_MinPktDuration_din  : out std_logic_vector(6-1 downto 0);
      |         sm_regAGC_AutoCorr_MinPktDuration_en   : out std_logic;
      |         -- 'regAGC_WSDAGCCtrl'
      |         sm_regAGC_WSDAGCCtrl_dout : in std_logic_vector(32-1 downto 0);
      |         sm_regAGC_WSDAGCCtrl_din  : out std_logic_vector(32-1 downto 0);
      |         sm_regAGC_WSDAGCCtrl_en   : out std_logic;
      |         -- 'regAGC_AutoCorr_RatioThresh'
      |         sm_regAGC_AutoCorr_RatioThresh_dout : in std_logic_vector(8-1 downto 0);
      |         sm_regAGC_AutoCorr_RatioThresh_din  : out std_logic_vector(8-1 downto 0);
      |         sm_regAGC_AutoCorr_RatioThresh_en   : out std_logic;
      |         -- 'regAGC_ManualRxVGA1_Gain'
      |         sm_regAGC_ManualRxVGA1_Gain_dout : in std_logic_vector(8-1 downto 0);
      |         sm_regAGC_ManualRxVGA1_Gain_din  : out std_logic_vector(8-1 downto 0);
      |         sm_regAGC_ManualRxVGA1_Gain_en   : out std_logic;
      |         -- 'regAGC_ManualRxLNA_Gain'
      |         sm_regAGC_ManualRxLNA_Gain_dout : in std_logic_vector(8-1 downto 0);
      |         sm_regAGC_ManualRxLNA_Gain_din  : out std_logic_vector(8-1 downto 0);
      |         sm_regAGC_ManualRxLNA_Gain_en   : out std_logic;
      |         -- 'regAGC_ManualRxVGA2_Gain'
      |         sm_regAGC_ManualRxVGA2_Gain_dout : in std_logic_vector(8-1 downto 0);
      |         sm_regAGC_ManualRxVGA2_Gain_din  : out std_logic_vector(8-1 downto 0);
      |         sm_regAGC_ManualRxVGA2_Gain_en   : out std_logic;
      |         -- 'regAGC_AutoCorr_LagTime'
      |         sm_regAGC_AutoCorr_LagTime_dout : in std_logic_vector(12-1 downto 0);
      |         sm_regAGC_AutoCorr_LagTime_din  : out std_logic_vector(12-1 downto 0);
      |         sm_regAGC_AutoCorr_LagTime_en   : out std_logic;
      |         -- 'regAGC_pktDetPwr_absoluteThreshold_dBm'
      |         sm_regAGC_pktDetPwr_absoluteThreshold_dBm_dout : in std_logic_vector(9-1 downto 0);
      |         sm_regAGC_pktDetPwr_absoluteThreshold_dBm_din  : out std_logic_vector(9-1 downto 0);
      |         sm_regAGC_pktDetPwr_absoluteThreshold_dBm_en   : out std_logic;
      |         -- 'regAGC_pktDetPwr_detectLag'
      |         sm_regAGC_pktDetPwr_detectLag_dout : in std_logic_vector(6-1 downto 0);
      |         sm_regAGC_pktDetPwr_detectLag_din  : out std_logic_vector(6-1 downto 0);
      |         sm_regAGC_pktDetPwr_detectLag_en   : out std_logic;
      |         -- 'regAGC_NumFineGainSteps'
      |         sm_regAGC_NumFineGainSteps_dout : in std_logic_vector(4-1 downto 0);
      |         sm_regAGC_NumFineGainSteps_din  : out std_logic_vector(4-1 downto 0);
      |         sm_regAGC_NumFineGainSteps_en   : out std_logic;
      |         -- 'regAGC_WSD_CCAThreshold_dBm'
      |         sm_regAGC_WSD_CCAThreshold_dBm_dout : in std_logic_vector(10-1 downto 0);
      |         sm_regAGC_WSD_CCAThreshold_dBm_din  : out std_logic_vector(10-1 downto 0);
      |         sm_regAGC_WSD_CCAThreshold_dBm_en   : out std_logic;
      |         -- 'regAGC_LongCorr_Threshold'
      |         sm_regAGC_LongCorr_Threshold_dout : in std_logic_vector(32-1 downto 0);
      |         sm_regAGC_LongCorr_Threshold_din  : out std_logic_vector(32-1 downto 0);
      |         sm_regAGC_LongCorr_Threshold_en   : out std_logic;
      |         -- 'regAGC_pktDetPwr_deltaThreshold_dBm'
      |         sm_regAGC_pktDetPwr_deltaThreshold_dBm_dout : in std_logic_vector(9-1 downto 0);
      |         sm_regAGC_pktDetPwr_deltaThreshold_dBm_din  : out std_logic_vector(9-1 downto 0);
      |         sm_regAGC_pktDetPwr_deltaThreshold_dBm_en   : out std_logic;
      |         -- 'regAGC_SPITIMINGFUDGE'
      |         sm_regAGC_SPITIMINGFUDGE_dout : in std_logic_vector(12-1 downto 0);
      |         sm_regAGC_SPITIMINGFUDGE_din  : out std_logic_vector(12-1 downto 0);
      |         sm_regAGC_SPITIMINGFUDGE_en   : out std_logic;
      |         -- 'From FIFO'
      |         -- 'To FIFO'
      |         -- 'Shared Memory'
      | 
      |         S_AXI_RLAST   : out std_logic;
      |         S_AXI_RID     : out std_logic_vector(C_S_AXI_ID_WIDTH-1 downto 0);
      |         S_AXI_RDATA   : out std_logic_vector(C_S_AXI_DATA_WIDTH-1 downto 0);
      |         S_AXI_RRESP   : out std_logic_vector(1 downto 0);
      |         S_AXI_RVALID  : out std_logic;
      |         S_AXI_RREADY  : in  std_logic
      |     );
      | end entity axi_sgiface;
      | 
      | architecture IMP of axi_sgiface is
      | 
      | -- Internal signals for write channel.
      | signal S_AXI_BVALID_i       : std_logic;
      | signal S_AXI_BID_i          : std_logic_vector(C_S_AXI_ID_WIDTH-1 downto 0);
      | signal S_AXI_WREADY_i       : std_logic;
      |   
      | -- Internal signals for read channels.
      | signal S_AXI_ARLEN_i        : std_logic_vector(C_S_AXI_ARLEN_WIDTH-1 downto 0);
      | signal S_AXI_RLAST_i        : std_logic;
      | signal S_AXI_RREADY_i       : std_logic;
      | signal S_AXI_RVALID_i       : std_logic;
      | signal S_AXI_RDATA_i        : std_logic_vector(C_S_AXI_DATA_WIDTH-1 downto 0);
      | signal S_AXI_RID_i          : std_logic_vector(C_S_AXI_ID_WIDTH-1 downto 0);
      | 
      | -- for read channel
      | signal read_bank_addr_i     : std_logic_vector(C_S_AXI_BANK_ADDR_LEN-1 downto 0);
      | signal read_linear_addr_i   : std_logic_vector(C_S_AXI_LINEAR_ADDR_LEN-1 downto 0);
      | -- for write channel
      | signal write_bank_addr_i    : std_logic_vector(C_S_AXI_BANK_ADDR_LEN-1 downto 0);
      | signal write_linear_addr_i  : std_logic_vector(C_S_AXI_LINEAR_ADDR_LEN-1 downto 0);
      | 
      | signal reg_bank_out_i       : std_logic_vector(C_S_AXI_DATA_WIDTH-1 downto 0);
      | signal fifo_bank_out_i      : std_logic_vector(C_S_AXI_DATA_WIDTH-1 downto 0);
      | signal shmem_bank_out_i     : std_logic_vector(C_S_AXI_DATA_WIDTH-1 downto 0);
      |     
      | -- 'From Register'
      | -- 'regSatDet_SaturationDetected'
      | signal sm_regSatDet_SaturationDetected_dout_i  : std_logic_vector(C_S_AXI_DATA_WIDTH-1 downto 0);
      | -- 'regWSD_RXGAIN_READ'
      | signal sm_regWSD_RXGAIN_READ_dout_i  : std_logic_vector(C_S_AXI_DATA_WIDTH-1 downto 0);
      | -- 'regWSD_RSSI'
      | signal sm_regWSD_RSSI_dout_i  : std_logic_vector(C_S_AXI_DATA_WIDTH-1 downto 0);
      | -- 'regWSD_meanPower'
      | signal sm_regWSD_meanPower_dout_i  : std_logic_vector(C_S_AXI_DATA_WIDTH-1 downto 0);
      | -- 'regWSD_MeanDC_Q'
      | signal sm_regWSD_MeanDC_Q_dout_i  : std_logic_vector(C_S_AXI_DATA_WIDTH-1 downto 0);
      | -- 'regWSD_MeanDC_I'
      | signal sm_regWSD_MeanDC_I_dout_i  : std_logic_vector(C_S_AXI_DATA_WIDTH-1 downto 0);
      | -- 'regWSD_RxLNAGain'
      | signal sm_regWSD_RxLNAGain_dout_i  : std_logic_vector(C_S_AXI_DATA_WIDTH-1 downto 0);
      | -- 'regWSD_RxVGA1Gain'
      | signal sm_regWSD_RxVGA1Gain_dout_i  : std_logic_vector(C_S_AXI_DATA_WIDTH-1 downto 0);
      | -- 'regWSD_RxVGA2Gain'
      | signal sm_regWSD_RxVGA2Gain_dout_i  : std_logic_vector(C_S_AXI_DATA_WIDTH-1 downto 0);
      | -- 'To Register'
      | -- 'regAGC_DefaultGainSettings'
      | signal sm_regAGC_DefaultGainSettings_din_i   : std_logic_vector(C_S_AXI_DATA_WIDTH-1 downto 0);
      | signal sm_regAGC_DefaultGainSettings_en_i    : std_logic;
      | signal sm_regAGC_DefaultGainSettings_dout_i  : std_logic_vector(C_S_AXI_DATA_WIDTH-1 downto 0);
      | -- 'regSPICtrl_SPIWriteDelay'
      | signal sm_regSPICtrl_SPIWriteDelay_din_i   : std_logic_vector(C_S_AXI_DATA_WIDTH-1 downto 0);
      | signal sm_regSPICtrl_SPIWriteDelay_en_i    : std_logic;
      | signal sm_regSPICtrl_SPIWriteDelay_dout_i  : std_logic_vector(C_S_AXI_DATA_WIDTH-1 downto 0);
      | -- 'regPwrMeas_AvgLength'
      | signal sm_regPwrMeas_AvgLength_din_i   : std_logic_vector(C_S_AXI_DATA_WIDTH-1 downto 0);
      | signal sm_regPwrMeas_AvgLength_en_i    : std_logic;
      | signal sm_regPwrMeas_AvgLength_dout_i  : std_logic_vector(C_S_AXI_DATA_WIDTH-1 downto 0);
      | -- 'regSatDet_SaturationMaxCount'
      | signal sm_regSatDet_SaturationMaxCount_din_i   : std_logic_vector(C_S_AXI_DATA_WIDTH-1 downto 0);
      | signal sm_regSatDet_SaturationMaxCount_en_i    : std_logic;
      | signal sm_regSatDet_SaturationMaxCount_dout_i  : std_logic_vector(C_S_AXI_DATA_WIDTH-1 downto 0);
      | -- 'regSatDet_NumSamples'
      | signal sm_regSatDet_NumSamples_din_i   : std_logic_vector(C_S_AXI_DATA_WIDTH-1 downto 0);
      | signal sm_regSatDet_NumSamples_en_i    : std_logic;
      | signal sm_regSatDet_NumSamples_dout_i  : std_logic_vector(C_S_AXI_DATA_WIDTH-1 downto 0);
      | -- 'regSatDet_SaturationThreshold'
      | signal sm_regSatDet_SaturationThreshold_din_i   : std_logic_vector(C_S_AXI_DATA_WIDTH-1 downto 0);
      | signal sm_regSatDet_SaturationThreshold_en_i    : std_logic;
      | signal sm_regSatDet_SaturationThreshold_dout_i  : std_logic_vector(C_S_AXI_DATA_WIDTH-1 downto 0);
      | -- 'regAGC_ExtPktDet_DelayCount'
      | signal sm_regAGC_ExtPktDet_DelayCount_din_i   : std_logic_vector(C_S_AXI_DATA_WIDTH-1 downto 0);
      | signal sm_regAGC_ExtPktDet_DelayCount_en_i    : std_logic;
      | signal sm_regAGC_ExtPktDet_DelayCount_dout_i  : std_logic_vector(C_S_AXI_DATA_WIDTH-1 downto 0);
      | -- 'regAGC_targetRxInputPwr'
      | signal sm_regAGC_targetRxInputPwr_din_i   : std_logic_vector(C_S_AXI_DATA_WIDTH-1 downto 0);
      | signal sm_regAGC_targetRxInputPwr_en_i    : std_logic;
      | signal sm_regAGC_targetRxInputPwr_dout_i  : std_logic_vector(C_S_AXI_DATA_WIDTH-1 downto 0);
      | -- 'regAGC_AutoCorr_MinPower'
      | signal sm_regAGC_AutoCorr_MinPower_din_i   : std_logic_vector(C_S_AXI_DATA_WIDTH-1 downto 0);
      | signal sm_regAGC_AutoCorr_MinPower_en_i    : std_logic;
      | signal sm_regAGC_AutoCorr_MinPower_dout_i  : std_logic_vector(C_S_AXI_DATA_WIDTH-1 downto 0);
      | -- 'regAGC_AutoCorr_MinPktDuration'
      | signal sm_regAGC_AutoCorr_MinPktDuration_din_i   : std_logic_vector(C_S_AXI_DATA_WIDTH-1 downto 0);
      | signal sm_regAGC_AutoCorr_MinPktDuration_en_i    : std_logic;
      | signal sm_regAGC_AutoCorr_MinPktDuration_dout_i  : std_logic_vector(C_S_AXI_DATA_WIDTH-1 downto 0);
      | -- 'regAGC_WSDAGCCtrl'
      | signal sm_regAGC_WSDAGCCtrl_din_i   : std_logic_vector(C_S_AXI_DATA_WIDTH-1 downto 0);
      | signal sm_regAGC_WSDAGCCtrl_en_i    : std_logic;
      | signal sm_regAGC_WSDAGCCtrl_dout_i  : std_logic_vector(C_S_AXI_DATA_WIDTH-1 downto 0);
      | -- 'regAGC_AutoCorr_RatioThresh'
      | signal sm_regAGC_AutoCorr_RatioThresh_din_i   : std_logic_vector(C_S_AXI_DATA_WIDTH-1 downto 0);
      | signal sm_regAGC_AutoCorr_RatioThresh_en_i    : std_logic;
      | signal sm_regAGC_AutoCorr_RatioThresh_dout_i  : std_logic_vector(C_S_AXI_DATA_WIDTH-1 downto 0);
      | -- 'regAGC_ManualRxVGA1_Gain'
      | signal sm_regAGC_ManualRxVGA1_Gain_din_i   : std_logic_vector(C_S_AXI_DATA_WIDTH-1 downto 0);
      | signal sm_regAGC_ManualRxVGA1_Gain_en_i    : std_logic;
      | signal sm_regAGC_ManualRxVGA1_Gain_dout_i  : std_logic_vector(C_S_AXI_DATA_WIDTH-1 downto 0);
      | -- 'regAGC_ManualRxLNA_Gain'
      | signal sm_regAGC_ManualRxLNA_Gain_din_i   : std_logic_vector(C_S_AXI_DATA_WIDTH-1 downto 0);
      | signal sm_regAGC_ManualRxLNA_Gain_en_i    : std_logic;
      | signal sm_regAGC_ManualRxLNA_Gain_dout_i  : std_logic_vector(C_S_AXI_DATA_WIDTH-1 downto 0);
      | -- 'regAGC_ManualRxVGA2_Gain'
      | signal sm_regAGC_ManualRxVGA2_Gain_din_i   : std_logic_vector(C_S_AXI_DATA_WIDTH-1 downto 0);
      | signal sm_regAGC_ManualRxVGA2_Gain_en_i    : std_logic;
      | signal sm_regAGC_ManualRxVGA2_Gain_dout_i  : std_logic_vector(C_S_AXI_DATA_WIDTH-1 downto 0);
      | -- 'regAGC_AutoCorr_LagTime'
      | signal sm_regAGC_AutoCorr_LagTime_din_i   : std_logic_vector(C_S_AXI_DATA_WIDTH-1 downto 0);
      | signal sm_regAGC_AutoCorr_LagTime_en_i    : std_logic;
      | signal sm_regAGC_AutoCorr_LagTime_dout_i  : std_logic_vector(C_S_AXI_DATA_WIDTH-1 downto 0);
      | -- 'regAGC_pktDetPwr_absoluteThreshold_dBm'
      | signal sm_regAGC_pktDetPwr_absoluteThreshold_dBm_din_i   : std_logic_vector(C_S_AXI_DATA_WIDTH-1 downto 0);
      | signal sm_regAGC_pktDetPwr_absoluteThreshold_dBm_en_i    : std_logic;
      | signal sm_regAGC_pktDetPwr_absoluteThreshold_dBm_dout_i  : std_logic_vector(C_S_AXI_DATA_WIDTH-1 downto 0);
      | -- 'regAGC_pktDetPwr_detectLag'
      | signal sm_regAGC_pktDetPwr_detectLag_din_i   : std_logic_vector(C_S_AXI_DATA_WIDTH-1 downto 0);
      | signal sm_regAGC_pktDetPwr_detectLag_en_i    : std_logic;
      | signal sm_regAGC_pktDetPwr_detectLag_dout_i  : std_logic_vector(C_S_AXI_DATA_WIDTH-1 downto 0);
      | -- 'regAGC_NumFineGainSteps'
      | signal sm_regAGC_NumFineGainSteps_din_i   : std_logic_vector(C_S_AXI_DATA_WIDTH-1 downto 0);
      | signal sm_regAGC_NumFineGainSteps_en_i    : std_logic;
      | signal sm_regAGC_NumFineGainSteps_dout_i  : std_logic_vector(C_S_AXI_DATA_WIDTH-1 downto 0);
      | -- 'regAGC_WSD_CCAThreshold_dBm'
      | signal sm_regAGC_WSD_CCAThreshold_dBm_din_i   : std_logic_vector(C_S_AXI_DATA_WIDTH-1 downto 0);
      | signal sm_regAGC_WSD_CCAThreshold_dBm_en_i    : std_logic;
      | signal sm_regAGC_WSD_CCAThreshold_dBm_dout_i  : std_logic_vector(C_S_AXI_DATA_WIDTH-1 downto 0);
      | -- 'regAGC_LongCorr_Threshold'
      | signal sm_regAGC_LongCorr_Threshold_din_i   : std_logic_vector(C_S_AXI_DATA_WIDTH-1 downto 0);
      | signal sm_regAGC_LongCorr_Threshold_en_i    : std_logic;
      | signal sm_regAGC_LongCorr_Threshold_dout_i  : std_logic_vector(C_S_AXI_DATA_WIDTH-1 downto 0);
      | -- 'regAGC_pktDetPwr_deltaThreshold_dBm'
      | signal sm_regAGC_pktDetPwr_deltaThreshold_dBm_din_i   : std_logic_vector(C_S_AXI_DATA_WIDTH-1 downto 0);
      | signal sm_regAGC_pktDetPwr_deltaThreshold_dBm_en_i    : std_logic;
      | signal sm_regAGC_pktDetPwr_deltaThreshold_dBm_dout_i  : std_logic_vector(C_S_AXI_DATA_WIDTH-1 downto 0);
      | -- 'regAGC_SPITIMINGFUDGE'
      | signal sm_regAGC_SPITIMINGFUDGE_din_i   : std_logic_vector(C_S_AXI_DATA_WIDTH-1 downto 0);
      | signal sm_regAGC_SPITIMINGFUDGE_en_i    : std_logic;
      | signal sm_regAGC_SPITIMINGFUDGE_dout_i  : std_logic_vector(C_S_AXI_DATA_WIDTH-1 downto 0);
      | -- 'From FIFO'
      | -- 'To FIFO'
      | -- 'Shared Memory'
      | 
      | type t_read_state is (IDLE, READ_PREP, READ_DATA);
      | signal read_state : t_read_state;
      | 
      | type t_write_state is (IDLE, WRITE_DATA, WRITE_RESPONSE);
      | signal write_state : t_write_state;
      | 
      | type t_memmap_state is (READ, WRITE);
      | signal memmap_state : t_memmap_state;
      | 
      | constant C_READ_PREP_DELAY : std_logic_vector(1 downto 0) := "11";
      | 
      | signal read_prep_counter : std_logic_vector(1 downto 0);
      | signal read_addr_counter : std_logic_vector(C_S_AXI_ARLEN_WIDTH-1 downto 0);
      | signal read_data_counter : std_logic_vector(C_S_AXI_ARLEN_WIDTH-1 downto 0);
      | 
      | -- enable of shared BRAMs
      | signal s_shram_en : std_logic;
      | 
      | signal write_addr_valid : std_logic;
      | signal write_ready : std_logic;
      | 
      | -- 're' of From/To FIFOs
      | signal s_fifo_re : std_logic;
      | -- 'we' of To FIFOs
      | signal s_fifo_we : std_logic;
      | 
      | begin
      | 
      | -- enable for 'Shared Memory' blocks
      | 
      | -- conversion to match with the data bus width
      | -- 'From Register'
      | -- 'regSatDet_SaturationDetected'
      | gen_sm_regSatDet_SaturationDetected_dout_i: if (1 < C_S_AXI_DATA_WIDTH) generate
      |     sm_regSatDet_SaturationDetected_dout_i(C_S_AXI_DATA_WIDTH-1 downto 1) <= (others => '0');
      | end generate gen_sm_regSatDet_SaturationDetected_dout_i;
      | sm_regSatDet_SaturationDetected_dout_i(1-1 downto 0) <= sm_regSatDet_SaturationDetected_dout;
      | -- 'regWSD_RXGAIN_READ'
      | gen_sm_regWSD_RXGAIN_READ_dout_i: if (9 < C_S_AXI_DATA_WIDTH) generate
      |     sm_regWSD_RXGAIN_READ_dout_i(C_S_AXI_DATA_WIDTH-1 downto 9) <= (others => '0');
      | end generate gen_sm_regWSD_RXGAIN_READ_dout_i;
      | sm_regWSD_RXGAIN_READ_dout_i(9-1 downto 0) <= sm_regWSD_RXGAIN_READ_dout;
      | -- 'regWSD_RSSI'
      | gen_sm_regWSD_RSSI_dout_i: if (10 < C_S_AXI_DATA_WIDTH) generate
      |     sm_regWSD_RSSI_dout_i(C_S_AXI_DATA_WIDTH-1 downto 10) <= (others => '0');
      | end generate gen_sm_regWSD_RSSI_dout_i;
      | sm_regWSD_RSSI_dout_i(10-1 downto 0) <= sm_regWSD_RSSI_dout;
      | -- 'regWSD_meanPower'
      | gen_sm_regWSD_meanPower_dout_i: if (9 < C_S_AXI_DATA_WIDTH) generate
      |     sm_regWSD_meanPower_dout_i(C_S_AXI_DATA_WIDTH-1 downto 9) <= (others => '0');
      | end generate gen_sm_regWSD_meanPower_dout_i;
      | sm_regWSD_meanPower_dout_i(9-1 downto 0) <= sm_regWSD_meanPower_dout;
      | -- 'regWSD_MeanDC_Q'
      | gen_sm_regWSD_MeanDC_Q_dout_i: if (12 < C_S_AXI_DATA_WIDTH) generate
      |     sm_regWSD_MeanDC_Q_dout_i(C_S_AXI_DATA_WIDTH-1 downto 12) <= (others => '0');
      | end generate gen_sm_regWSD_MeanDC_Q_dout_i;
      | sm_regWSD_MeanDC_Q_dout_i(12-1 downto 0) <= sm_regWSD_MeanDC_Q_dout;
      | -- 'regWSD_MeanDC_I'
      | gen_sm_regWSD_MeanDC_I_dout_i: if (12 < C_S_AXI_DATA_WIDTH) generate
      |     sm_regWSD_MeanDC_I_dout_i(C_S_AXI_DATA_WIDTH-1 downto 12) <= (others => '0');
      | end generate gen_sm_regWSD_MeanDC_I_dout_i;
      | sm_regWSD_MeanDC_I_dout_i(12-1 downto 0) <= sm_regWSD_MeanDC_I_dout;
      | -- 'regWSD_RxLNAGain'
      | gen_sm_regWSD_RxLNAGain_dout_i: if (8 < C_S_AXI_DATA_WIDTH) generate
      |     sm_regWSD_RxLNAGain_dout_i(C_S_AXI_DATA_WIDTH-1 downto 8) <= (others => '0');
      | end generate gen_sm_regWSD_RxLNAGain_dout_i;
      | sm_regWSD_RxLNAGain_dout_i(8-1 downto 0) <= sm_regWSD_RxLNAGain_dout;
      | -- 'regWSD_RxVGA1Gain'
      | gen_sm_regWSD_RxVGA1Gain_dout_i: if (8 < C_S_AXI_DATA_WIDTH) generate
      |     sm_regWSD_RxVGA1Gain_dout_i(C_S_AXI_DATA_WIDTH-1 downto 8) <= (others => '0');
      | end generate gen_sm_regWSD_RxVGA1Gain_dout_i;
      | sm_regWSD_RxVGA1Gain_dout_i(8-1 downto 0) <= sm_regWSD_RxVGA1Gain_dout;
      | -- 'regWSD_RxVGA2Gain'
      | gen_sm_regWSD_RxVGA2Gain_dout_i: if (8 < C_S_AXI_DATA_WIDTH) generate
      |     sm_regWSD_RxVGA2Gain_dout_i(C_S_AXI_DATA_WIDTH-1 downto 8) <= (others => '0');
      | end generate gen_sm_regWSD_RxVGA2Gain_dout_i;
      | sm_regWSD_RxVGA2Gain_dout_i(8-1 downto 0) <= sm_regWSD_RxVGA2Gain_dout;
      | -- 'To Register'
      | -- 'regAGC_DefaultGainSettings'
      | sm_regAGC_DefaultGainSettings_din     <= sm_regAGC_DefaultGainSettings_din_i(32-1 downto 0);
      | sm_regAGC_DefaultGainSettings_en      <= sm_regAGC_DefaultGainSettings_en_i;
      | gen_sm_regAGC_DefaultGainSettings_dout_i: if (32 < C_S_AXI_DATA_WIDTH) generate
      |     sm_regAGC_DefaultGainSettings_dout_i(C_S_AXI_DATA_WIDTH-1 downto 32) <= (others => '0');
      | end generate gen_sm_regAGC_DefaultGainSettings_dout_i;
      | sm_regAGC_DefaultGainSettings_dout_i(32-1 downto 0) <= sm_regAGC_DefaultGainSettings_dout;
      | -- 'regSPICtrl_SPIWriteDelay'
      | sm_regSPICtrl_SPIWriteDelay_din     <= sm_regSPICtrl_SPIWriteDelay_din_i(8-1 downto 0);
      | sm_regSPICtrl_SPIWriteDelay_en      <= sm_regSPICtrl_SPIWriteDelay_en_i;
      | gen_sm_regSPICtrl_SPIWriteDelay_dout_i: if (8 < C_S_AXI_DATA_WIDTH) generate
      |     sm_regSPICtrl_SPIWriteDelay_dout_i(C_S_AXI_DATA_WIDTH-1 downto 8) <= (others => '0');
      | end generate gen_sm_regSPICtrl_SPIWriteDelay_dout_i;
      | sm_regSPICtrl_SPIWriteDelay_dout_i(8-1 downto 0) <= sm_regSPICtrl_SPIWriteDelay_dout;
      | -- 'regPwrMeas_AvgLength'
      | sm_regPwrMeas_AvgLength_din     <= sm_regPwrMeas_AvgLength_din_i(7-1 downto 0);
      | sm_regPwrMeas_AvgLength_en      <= sm_regPwrMeas_AvgLength_en_i;
      | gen_sm_regPwrMeas_AvgLength_dout_i: if (7 < C_S_AXI_DATA_WIDTH) generate
      |     sm_regPwrMeas_AvgLength_dout_i(C_S_AXI_DATA_WIDTH-1 downto 7) <= (others => '0');
      | end generate gen_sm_regPwrMeas_AvgLength_dout_i;
      | sm_regPwrMeas_AvgLength_dout_i(7-1 downto 0) <= sm_regPwrMeas_AvgLength_dout;
      | -- 'regSatDet_SaturationMaxCount'
      | sm_regSatDet_SaturationMaxCount_din     <= sm_regSatDet_SaturationMaxCount_din_i(6-1 downto 0);
      | sm_regSatDet_SaturationMaxCount_en      <= sm_regSatDet_SaturationMaxCount_en_i;
      | gen_sm_regSatDet_SaturationMaxCount_dout_i: if (6 < C_S_AXI_DATA_WIDTH) generate
      |     sm_regSatDet_SaturationMaxCount_dout_i(C_S_AXI_DATA_WIDTH-1 downto 6) <= (others => '0');
      | end generate gen_sm_regSatDet_SaturationMaxCount_dout_i;
      | sm_regSatDet_SaturationMaxCount_dout_i(6-1 downto 0) <= sm_regSatDet_SaturationMaxCount_dout;
      | -- 'regSatDet_NumSamples'
      | sm_regSatDet_NumSamples_din     <= sm_regSatDet_NumSamples_din_i(5-1 downto 0);
      | sm_regSatDet_NumSamples_en      <= sm_regSatDet_NumSamples_en_i;
      | gen_sm_regSatDet_NumSamples_dout_i: if (5 < C_S_AXI_DATA_WIDTH) generate
      |     sm_regSatDet_NumSamples_dout_i(C_S_AXI_DATA_WIDTH-1 downto 5) <= (others => '0');
      | end generate gen_sm_regSatDet_NumSamples_dout_i;
      | sm_regSatDet_NumSamples_dout_i(5-1 downto 0) <= sm_regSatDet_NumSamples_dout;
      | -- 'regSatDet_SaturationThreshold'
      | sm_regSatDet_SaturationThreshold_din     <= sm_regSatDet_SaturationThreshold_din_i(14-1 downto 0);
      | sm_regSatDet_SaturationThreshold_en      <= sm_regSatDet_SaturationThreshold_en_i;
      | gen_sm_regSatDet_SaturationThreshold_dout_i: if (14 < C_S_AXI_DATA_WIDTH) generate
      |     sm_regSatDet_SaturationThreshold_dout_i(C_S_AXI_DATA_WIDTH-1 downto 14) <= (others => '0');
      | end generate gen_sm_regSatDet_SaturationThreshold_dout_i;
      | sm_regSatDet_SaturationThreshold_dout_i(14-1 downto 0) <= sm_regSatDet_SaturationThreshold_dout;
      | -- 'regAGC_ExtPktDet_DelayCount'
      | sm_regAGC_ExtPktDet_DelayCount_din     <= sm_regAGC_ExtPktDet_DelayCount_din_i(32-1 downto 0);
      | sm_regAGC_ExtPktDet_DelayCount_en      <= sm_regAGC_ExtPktDet_DelayCount_en_i;
      | gen_sm_regAGC_ExtPktDet_DelayCount_dout_i: if (32 < C_S_AXI_DATA_WIDTH) generate
      |     sm_regAGC_ExtPktDet_DelayCount_dout_i(C_S_AXI_DATA_WIDTH-1 downto 32) <= (others => '0');
      | end generate gen_sm_regAGC_ExtPktDet_DelayCount_dout_i;
      | sm_regAGC_ExtPktDet_DelayCount_dout_i(32-1 downto 0) <= sm_regAGC_ExtPktDet_DelayCount_dout;
      | -- 'regAGC_targetRxInputPwr'
      | sm_regAGC_targetRxInputPwr_din     <= sm_regAGC_targetRxInputPwr_din_i(9-1 downto 0);
      | sm_regAGC_targetRxInputPwr_en      <= sm_regAGC_targetRxInputPwr_en_i;
      | gen_sm_regAGC_targetRxInputPwr_dout_i: if (9 < C_S_AXI_DATA_WIDTH) generate
      |     sm_regAGC_targetRxInputPwr_dout_i(C_S_AXI_DATA_WIDTH-1 downto 9) <= (others => '0');
      | end generate gen_sm_regAGC_targetRxInputPwr_dout_i;
      | sm_regAGC_targetRxInputPwr_dout_i(9-1 downto 0) <= sm_regAGC_targetRxInputPwr_dout;
      | -- 'regAGC_AutoCorr_MinPower'
      | sm_regAGC_AutoCorr_MinPower_din     <= sm_regAGC_AutoCorr_MinPower_din_i(16-1 downto 0);
      | sm_regAGC_AutoCorr_MinPower_en      <= sm_regAGC_AutoCorr_MinPower_en_i;
      | gen_sm_regAGC_AutoCorr_MinPower_dout_i: if (16 < C_S_AXI_DATA_WIDTH) generate
      |     sm_regAGC_AutoCorr_MinPower_dout_i(C_S_AXI_DATA_WIDTH-1 downto 16) <= (others => '0');
      | end generate gen_sm_regAGC_AutoCorr_MinPower_dout_i;
      | sm_regAGC_AutoCorr_MinPower_dout_i(16-1 downto 0) <= sm_regAGC_AutoCorr_MinPower_dout;
      | -- 'regAGC_AutoCorr_MinPktDuration'
      | sm_regAGC_AutoCorr_MinPktDuration_din     <= sm_regAGC_AutoCorr_MinPktDuration_din_i(6-1 downto 0);
      | sm_regAGC_AutoCorr_MinPktDuration_en      <= sm_regAGC_AutoCorr_MinPktDuration_en_i;
      | gen_sm_regAGC_AutoCorr_MinPktDuration_dout_i: if (6 < C_S_AXI_DATA_WIDTH) generate
      |     sm_regAGC_AutoCorr_MinPktDuration_dout_i(C_S_AXI_DATA_WIDTH-1 downto 6) <= (others => '0');
      | end generate gen_sm_regAGC_AutoCorr_MinPktDuration_dout_i;
      | sm_regAGC_AutoCorr_MinPktDuration_dout_i(6-1 downto 0) <= sm_regAGC_AutoCorr_MinPktDuration_dout;
      | -- 'regAGC_WSDAGCCtrl'
      | sm_regAGC_WSDAGCCtrl_din     <= sm_regAGC_WSDAGCCtrl_din_i(32-1 downto 0);
      | sm_regAGC_WSDAGCCtrl_en      <= sm_regAGC_WSDAGCCtrl_en_i;
      | gen_sm_regAGC_WSDAGCCtrl_dout_i: if (32 < C_S_AXI_DATA_WIDTH) generate
      |     sm_regAGC_WSDAGCCtrl_dout_i(C_S_AXI_DATA_WIDTH-1 downto 32) <= (others => '0');
      | end generate gen_sm_regAGC_WSDAGCCtrl_dout_i;
      | sm_regAGC_WSDAGCCtrl_dout_i(32-1 downto 0) <= sm_regAGC_WSDAGCCtrl_dout;
      | -- 'regAGC_AutoCorr_RatioThresh'
      | sm_regAGC_AutoCorr_RatioThresh_din     <= sm_regAGC_AutoCorr_RatioThresh_din_i(8-1 downto 0);
      | sm_regAGC_AutoCorr_RatioThresh_en      <= sm_regAGC_AutoCorr_RatioThresh_en_i;
      | gen_sm_regAGC_AutoCorr_RatioThresh_dout_i: if (8 < C_S_AXI_DATA_WIDTH) generate
      |     sm_regAGC_AutoCorr_RatioThresh_dout_i(C_S_AXI_DATA_WIDTH-1 downto 8) <= (others => '0');
      | end generate gen_sm_regAGC_AutoCorr_RatioThresh_dout_i;
      | sm_regAGC_AutoCorr_RatioThresh_dout_i(8-1 downto 0) <= sm_regAGC_AutoCorr_RatioThresh_dout;
      | -- 'regAGC_ManualRxVGA1_Gain'
      | sm_regAGC_ManualRxVGA1_Gain_din     <= sm_regAGC_ManualRxVGA1_Gain_din_i(8-1 downto 0);
      | sm_regAGC_ManualRxVGA1_Gain_en      <= sm_regAGC_ManualRxVGA1_Gain_en_i;
      | gen_sm_regAGC_ManualRxVGA1_Gain_dout_i: if (8 < C_S_AXI_DATA_WIDTH) generate
      |     sm_regAGC_ManualRxVGA1_Gain_dout_i(C_S_AXI_DATA_WIDTH-1 downto 8) <= (others => '0');
      | end generate gen_sm_regAGC_ManualRxVGA1_Gain_dout_i;
      | sm_regAGC_ManualRxVGA1_Gain_dout_i(8-1 downto 0) <= sm_regAGC_ManualRxVGA1_Gain_dout;
      | -- 'regAGC_ManualRxLNA_Gain'
      | sm_regAGC_ManualRxLNA_Gain_din     <= sm_regAGC_ManualRxLNA_Gain_din_i(8-1 downto 0);
      | sm_regAGC_ManualRxLNA_Gain_en      <= sm_regAGC_ManualRxLNA_Gain_en_i;
      | gen_sm_regAGC_ManualRxLNA_Gain_dout_i: if (8 < C_S_AXI_DATA_WIDTH) generate
      |     sm_regAGC_ManualRxLNA_Gain_dout_i(C_S_AXI_DATA_WIDTH-1 downto 8) <= (others => '0');
      | end generate gen_sm_regAGC_ManualRxLNA_Gain_dout_i;
      | sm_regAGC_ManualRxLNA_Gain_dout_i(8-1 downto 0) <= sm_regAGC_ManualRxLNA_Gain_dout;
      | -- 'regAGC_ManualRxVGA2_Gain'
      | sm_regAGC_ManualRxVGA2_Gain_din     <= sm_regAGC_ManualRxVGA2_Gain_din_i(8-1 downto 0);
      | sm_regAGC_ManualRxVGA2_Gain_en      <= sm_regAGC_ManualRxVGA2_Gain_en_i;
      | gen_sm_regAGC_ManualRxVGA2_Gain_dout_i: if (8 < C_S_AXI_DATA_WIDTH) generate
      |     sm_regAGC_ManualRxVGA2_Gain_dout_i(C_S_AXI_DATA_WIDTH-1 downto 8) <= (others => '0');
      | end generate gen_sm_regAGC_ManualRxVGA2_Gain_dout_i;
      | sm_regAGC_ManualRxVGA2_Gain_dout_i(8-1 downto 0) <= sm_regAGC_ManualRxVGA2_Gain_dout;
      | -- 'regAGC_AutoCorr_LagTime'
      | sm_regAGC_AutoCorr_LagTime_din     <= sm_regAGC_AutoCorr_LagTime_din_i(12-1 downto 0);
      | sm_regAGC_AutoCorr_LagTime_en      <= sm_regAGC_AutoCorr_LagTime_en_i;
      | gen_sm_regAGC_AutoCorr_LagTime_dout_i: if (12 < C_S_AXI_DATA_WIDTH) generate
      |     sm_regAGC_AutoCorr_LagTime_dout_i(C_S_AXI_DATA_WIDTH-1 downto 12) <= (others => '0');
      | end generate gen_sm_regAGC_AutoCorr_LagTime_dout_i;
      | sm_regAGC_AutoCorr_LagTime_dout_i(12-1 downto 0) <= sm_regAGC_AutoCorr_LagTime_dout;
      | -- 'regAGC_pktDetPwr_absoluteThreshold_dBm'
      | sm_regAGC_pktDetPwr_absoluteThreshold_dBm_din     <= sm_regAGC_pktDetPwr_absoluteThreshold_dBm_din_i(9-1 downto 0);
      | sm_regAGC_pktDetPwr_absoluteThreshold_dBm_en      <= sm_regAGC_pktDetPwr_absoluteThreshold_dBm_en_i;
      | gen_sm_regAGC_pktDetPwr_absoluteThreshold_dBm_dout_i: if (9 < C_S_AXI_DATA_WIDTH) generate
      |     sm_regAGC_pktDetPwr_absoluteThreshold_dBm_dout_i(C_S_AXI_DATA_WIDTH-1 downto 9) <= (others => '0');
      | end generate gen_sm_regAGC_pktDetPwr_absoluteThreshold_dBm_dout_i;
      | sm_regAGC_pktDetPwr_absoluteThreshold_dBm_dout_i(9-1 downto 0) <= sm_regAGC_pktDetPwr_absoluteThreshold_dBm_dout;
      | -- 'regAGC_pktDetPwr_detectLag'
      | sm_regAGC_pktDetPwr_detectLag_din     <= sm_regAGC_pktDetPwr_detectLag_din_i(6-1 downto 0);
      | sm_regAGC_pktDetPwr_detectLag_en      <= sm_regAGC_pktDetPwr_detectLag_en_i;
      | gen_sm_regAGC_pktDetPwr_detectLag_dout_i: if (6 < C_S_AXI_DATA_WIDTH) generate
      |     sm_regAGC_pktDetPwr_detectLag_dout_i(C_S_AXI_DATA_WIDTH-1 downto 6) <= (others => '0');
      | end generate gen_sm_regAGC_pktDetPwr_detectLag_dout_i;
      | sm_regAGC_pktDetPwr_detectLag_dout_i(6-1 downto 0) <= sm_regAGC_pktDetPwr_detectLag_dout;
      | -- 'regAGC_NumFineGainSteps'
      | sm_regAGC_NumFineGainSteps_din     <= sm_regAGC_NumFineGainSteps_din_i(4-1 downto 0);
      | sm_regAGC_NumFineGainSteps_en      <= sm_regAGC_NumFineGainSteps_en_i;
      | gen_sm_regAGC_NumFineGainSteps_dout_i: if (4 < C_S_AXI_DATA_WIDTH) generate
      |     sm_regAGC_NumFineGainSteps_dout_i(C_S_AXI_DATA_WIDTH-1 downto 4) <= (others => '0');
      | end generate gen_sm_regAGC_NumFineGainSteps_dout_i;
      | sm_regAGC_NumFineGainSteps_dout_i(4-1 downto 0) <= sm_regAGC_NumFineGainSteps_dout;
      | -- 'regAGC_WSD_CCAThreshold_dBm'
      | sm_regAGC_WSD_CCAThreshold_dBm_din     <= sm_regAGC_WSD_CCAThreshold_dBm_din_i(10-1 downto 0);
      | sm_regAGC_WSD_CCAThreshold_dBm_en      <= sm_regAGC_WSD_CCAThreshold_dBm_en_i;
      | gen_sm_regAGC_WSD_CCAThreshold_dBm_dout_i: if (10 < C_S_AXI_DATA_WIDTH) generate
      |     sm_regAGC_WSD_CCAThreshold_dBm_dout_i(C_S_AXI_DATA_WIDTH-1 downto 10) <= (others => '0');
      | end generate gen_sm_regAGC_WSD_CCAThreshold_dBm_dout_i;
      | sm_regAGC_WSD_CCAThreshold_dBm_dout_i(10-1 downto 0) <= sm_regAGC_WSD_CCAThreshold_dBm_dout;
      | -- 'regAGC_LongCorr_Threshold'
      | sm_regAGC_LongCorr_Threshold_din     <= sm_regAGC_LongCorr_Threshold_din_i(32-1 downto 0);
      | sm_regAGC_LongCorr_Threshold_en      <= sm_regAGC_LongCorr_Threshold_en_i;
      | gen_sm_regAGC_LongCorr_Threshold_dout_i: if (32 < C_S_AXI_DATA_WIDTH) generate
      |     sm_regAGC_LongCorr_Threshold_dout_i(C_S_AXI_DATA_WIDTH-1 downto 32) <= (others => '0');
      | end generate gen_sm_regAGC_LongCorr_Threshold_dout_i;
      | sm_regAGC_LongCorr_Threshold_dout_i(32-1 downto 0) <= sm_regAGC_LongCorr_Threshold_dout;
      | -- 'regAGC_pktDetPwr_deltaThreshold_dBm'
      | sm_regAGC_pktDetPwr_deltaThreshold_dBm_din     <= sm_regAGC_pktDetPwr_deltaThreshold_dBm_din_i(9-1 downto 0);
      | sm_regAGC_pktDetPwr_deltaThreshold_dBm_en      <= sm_regAGC_pktDetPwr_deltaThreshold_dBm_en_i;
      | gen_sm_regAGC_pktDetPwr_deltaThreshold_dBm_dout_i: if (9 < C_S_AXI_DATA_WIDTH) generate
      |     sm_regAGC_pktDetPwr_deltaThreshold_dBm_dout_i(C_S_AXI_DATA_WIDTH-1 downto 9) <= (others => '0');
      | end generate gen_sm_regAGC_pktDetPwr_deltaThreshold_dBm_dout_i;
      | sm_regAGC_pktDetPwr_deltaThreshold_dBm_dout_i(9-1 downto 0) <= sm_regAGC_pktDetPwr_deltaThreshold_dBm_dout;
      | -- 'regAGC_SPITIMINGFUDGE'
      | sm_regAGC_SPITIMINGFUDGE_din     <= sm_regAGC_SPITIMINGFUDGE_din_i(12-1 downto 0);
      | sm_regAGC_SPITIMINGFUDGE_en      <= sm_regAGC_SPITIMINGFUDGE_en_i;
      | gen_sm_regAGC_SPITIMINGFUDGE_dout_i: if (12 < C_S_AXI_DATA_WIDTH) generate
      |     sm_regAGC_SPITIMINGFUDGE_dout_i(C_S_AXI_DATA_WIDTH-1 downto 12) <= (others => '0');
      | end generate gen_sm_regAGC_SPITIMINGFUDGE_dout_i;
      | sm_regAGC_SPITIMINGFUDGE_dout_i(12-1 downto 0) <= sm_regAGC_SPITIMINGFUDGE_dout;
      | -- 'From FIFO'
      | -- 'To FIFO'
      | -- 'Shared Memory'
      | 
      | ReadWriteSelect: process(memmap_state) is begin
      |     if (memmap_state = READ) then
      |     else
      |     end if;
      | end process ReadWriteSelect;
      | 
      | -----------------------------------------------------------------------------
      | -- address for 'Shared Memory'
      | -----------------------------------------------------------------------------
      | SharedMemory_Addr_ResetN : process(AXI_AClk) is begin
      |     if (AXI_AClk'event and AXI_AClk = '1') then
      |         if (AXI_AResetN = '0') then
      |             memmap_state <= READ;
      |         else
      |             if (S_AXI_AWVALID = '1') then
      |                 -- write operation
      |                 memmap_state <= WRITE;
      |             elsif (S_AXI_ARVALID = '1') then
      |                 -- read operation
      |                 memmap_state <= READ;
      |             end if;
      |         end if;
      |     end if;
      | end process SharedMemory_Addr_ResetN;
      | 
      | -----------------------------------------------------------------------------
      | -- WRITE Command Control
      | -----------------------------------------------------------------------------
      | S_AXI_BID     <= S_AXI_BID_i;
      | S_AXI_BVALID  <= S_AXI_BVALID_i;
      | S_AXI_WREADY  <= S_AXI_WREADY_i;
      | -- No error checking
      | S_AXI_BRESP  <= (others=>'0');
      | 
      | PROC_AWREADY_ACK: process(read_state, write_state, S_AXI_ARVALID, S_AXI_AWVALID) is begin
      |     if (write_state = IDLE and S_AXI_AWVALID = '1' and read_state = IDLE) then
      |         S_AXI_AWREADY <= S_AXI_AWVALID;
      |     else
      |         S_AXI_AWREADY <= '0';
      |     end if;
      | end process PROC_AWREADY_ACK;
      | 
      | Cmd_Decode_Write: process(AXI_AClk) is begin
      |     if (AXI_AClk'event and AXI_AClk = '1') then
      |         if (AXI_AResetN = '0') then
      |             write_addr_valid    <= '0';
      |             write_ready         <= '0';
      |             s_fifo_we           <= '0';
      |             S_AXI_BVALID_i      <= '0';
      |             S_AXI_BID_i         <= (others => '0');
      |             write_bank_addr_i   <= (others => '0');
      |             write_linear_addr_i <= (others => '0');
      |         else
      |             if (write_state = IDLE) then
      |                 if (S_AXI_AWVALID = '1' and read_state = IDLE) then
      |                     -- reflect awid
      |                     S_AXI_BID_i <= S_AXI_AWID;
      | 
      |                     -- latch bank and linear addresses
      |                     write_bank_addr_i   <= S_AXI_AWADDR(C_S_AXI_TOTAL_ADDR_LEN-1 downto C_S_AXI_LINEAR_ADDR_LEN+2);
      |                     write_linear_addr_i <= S_AXI_AWADDR(C_S_AXI_LINEAR_ADDR_LEN+1 downto 2);
      |                     write_addr_valid <= '1';
      |                     s_fifo_we <= '1';
      | 
      |                     -- write state transition
      |                     write_state <= WRITE_DATA;
      |                 end if;
      |             elsif (write_state = WRITE_DATA) then
      |                 write_ready <= '1';
      |                 s_fifo_we <= '0';
      |                 write_addr_valid <= S_AXI_WVALID;
      |                 
      |                 if (S_AXI_WVALID = '1' and write_ready = '1') then
      |                     write_linear_addr_i <= Std_Logic_Vector(unsigned(write_linear_addr_i) + 1);
      |                 end if;
      | 
      |                 if (S_AXI_WLAST = '1' and write_ready = '1') then
      |                     -- start responding through B channel upon the last write data sample
      |                     S_AXI_BVALID_i <= '1';
      |                     -- write data is over
      |                     write_addr_valid <= '0';
      |                     write_ready <= '0';
      |                     -- write state transition
      |                     write_state <= WRITE_RESPONSE;
      |                 end if;
      |             elsif (write_state = WRITE_RESPONSE) then
      | 
      |                 if (S_AXI_BREADY = '1') then
      |                     -- write respond is over
      |                     S_AXI_BVALID_i <= '0';
      |                     S_AXI_BID_i <= (others => '0');
      | 
      |                     -- write state transition
      |                     write_state <= IDLE;
      |                 end if;
      |             end if;
      |         end if;
      |     end if;
      | end process Cmd_Decode_Write;
      | 
      | Write_Linear_Addr_Decode : process(AXI_AClk) is 
      | 
      | begin
      |     if (AXI_AClk'event and AXI_AClk = '1') then
      |         if (AXI_AResetN = '0') then
      |             -- 'To Register'
      |             -- regAGC_DefaultGainSettings din/en
      |             sm_regAGC_DefaultGainSettings_din_i <= (others => '0');
      |             sm_regAGC_DefaultGainSettings_en_i <= '0';
      |             -- regSPICtrl_SPIWriteDelay din/en
      |             sm_regSPICtrl_SPIWriteDelay_din_i <= (others => '0');
      |             sm_regSPICtrl_SPIWriteDelay_en_i <= '0';
      |             -- regPwrMeas_AvgLength din/en
      |             sm_regPwrMeas_AvgLength_din_i <= (others => '0');
      |             sm_regPwrMeas_AvgLength_en_i <= '0';
      |             -- regSatDet_SaturationMaxCount din/en
      |             sm_regSatDet_SaturationMaxCount_din_i <= (others => '0');
      |             sm_regSatDet_SaturationMaxCount_en_i <= '0';
      |             -- regSatDet_NumSamples din/en
      |             sm_regSatDet_NumSamples_din_i <= (others => '0');
      |             sm_regSatDet_NumSamples_en_i <= '0';
      |             -- regSatDet_SaturationThreshold din/en
      |             sm_regSatDet_SaturationThreshold_din_i <= (others => '0');
      |             sm_regSatDet_SaturationThreshold_en_i <= '0';
      |             -- regAGC_ExtPktDet_DelayCount din/en
      |             sm_regAGC_ExtPktDet_DelayCount_din_i <= (others => '0');
      |             sm_regAGC_ExtPktDet_DelayCount_en_i <= '0';
      |             -- regAGC_targetRxInputPwr din/en
      |             sm_regAGC_targetRxInputPwr_din_i <= (others => '0');
      |             sm_regAGC_targetRxInputPwr_en_i <= '0';
      |             -- regAGC_AutoCorr_MinPower din/en
      |             sm_regAGC_AutoCorr_MinPower_din_i <= (others => '0');
      |             sm_regAGC_AutoCorr_MinPower_en_i <= '0';
      |             -- regAGC_AutoCorr_MinPktDuration din/en
      |             sm_regAGC_AutoCorr_MinPktDuration_din_i <= (others => '0');
      |             sm_regAGC_AutoCorr_MinPktDuration_en_i <= '0';
      |             -- regAGC_WSDAGCCtrl din/en
      |             sm_regAGC_WSDAGCCtrl_din_i <= (others => '0');
      |             sm_regAGC_WSDAGCCtrl_en_i <= '0';
      |             -- regAGC_AutoCorr_RatioThresh din/en
      |             sm_regAGC_AutoCorr_RatioThresh_din_i <= (others => '0');
      |             sm_regAGC_AutoCorr_RatioThresh_en_i <= '0';
      |             -- regAGC_ManualRxVGA1_Gain din/en
      |             sm_regAGC_ManualRxVGA1_Gain_din_i <= (others => '0');
      |             sm_regAGC_ManualRxVGA1_Gain_en_i <= '0';
      |             -- regAGC_ManualRxLNA_Gain din/en
      |             sm_regAGC_ManualRxLNA_Gain_din_i <= (others => '0');
      |             sm_regAGC_ManualRxLNA_Gain_en_i <= '0';
      |             -- regAGC_ManualRxVGA2_Gain din/en
      |             sm_regAGC_ManualRxVGA2_Gain_din_i <= (others => '0');
      |             sm_regAGC_ManualRxVGA2_Gain_en_i <= '0';
      |             -- regAGC_AutoCorr_LagTime din/en
      |             sm_regAGC_AutoCorr_LagTime_din_i <= (others => '0');
      |             sm_regAGC_AutoCorr_LagTime_en_i <= '0';
      |             -- regAGC_pktDetPwr_absoluteThreshold_dBm din/en
      |             sm_regAGC_pktDetPwr_absoluteThreshold_dBm_din_i <= (others => '0');
      |             sm_regAGC_pktDetPwr_absoluteThreshold_dBm_en_i <= '0';
      |             -- regAGC_pktDetPwr_detectLag din/en
      |             sm_regAGC_pktDetPwr_detectLag_din_i <= (others => '0');
      |             sm_regAGC_pktDetPwr_detectLag_en_i <= '0';
      |             -- regAGC_NumFineGainSteps din/en
      |             sm_regAGC_NumFineGainSteps_din_i <= (others => '0');
      |             sm_regAGC_NumFineGainSteps_en_i <= '0';
      |             -- regAGC_WSD_CCAThreshold_dBm din/en
      |             sm_regAGC_WSD_CCAThreshold_dBm_din_i <= (others => '0');
      |             sm_regAGC_WSD_CCAThreshold_dBm_en_i <= '0';
      |             -- regAGC_LongCorr_Threshold din/en
      |             sm_regAGC_LongCorr_Threshold_din_i <= (others => '0');
      |             sm_regAGC_LongCorr_Threshold_en_i <= '0';
      |             -- regAGC_pktDetPwr_deltaThreshold_dBm din/en
      |             sm_regAGC_pktDetPwr_deltaThreshold_dBm_din_i <= (others => '0');
      |             sm_regAGC_pktDetPwr_deltaThreshold_dBm_en_i <= '0';
      |             -- regAGC_SPITIMINGFUDGE din/en
      |             sm_regAGC_SPITIMINGFUDGE_din_i <= (others => '0');
      |             sm_regAGC_SPITIMINGFUDGE_en_i <= '0';
      |             -- 'To FIFO'
      |             -- 'Shared Memory'
      |         else
      |             -- default assignments
      | 
      |             -- 'To Register'
      |             if (unsigned(write_bank_addr_i) = 2) then
      |                 if (unsigned(write_linear_addr_i) = 0) then
      |                     -- regAGC_DefaultGainSettings din/en
      |                     sm_regAGC_DefaultGainSettings_din_i <= S_AXI_WDATA;
      |                     sm_regAGC_DefaultGainSettings_en_i  <= write_addr_valid;
      |                 elsif (unsigned(write_linear_addr_i) = 1) then
      |                     -- regSPICtrl_SPIWriteDelay din/en
      |                     sm_regSPICtrl_SPIWriteDelay_din_i <= S_AXI_WDATA;
      |                     sm_regSPICtrl_SPIWriteDelay_en_i  <= write_addr_valid;
      |                 elsif (unsigned(write_linear_addr_i) = 2) then
      |                     -- regPwrMeas_AvgLength din/en
      |                     sm_regPwrMeas_AvgLength_din_i <= S_AXI_WDATA;
      |                     sm_regPwrMeas_AvgLength_en_i  <= write_addr_valid;
      |                 elsif (unsigned(write_linear_addr_i) = 3) then
      |                     -- regSatDet_SaturationMaxCount din/en
      |                     sm_regSatDet_SaturationMaxCount_din_i <= S_AXI_WDATA;
      |                     sm_regSatDet_SaturationMaxCount_en_i  <= write_addr_valid;
      |                 elsif (unsigned(write_linear_addr_i) = 4) then
      |                     -- regSatDet_NumSamples din/en
      |                     sm_regSatDet_NumSamples_din_i <= S_AXI_WDATA;
      |                     sm_regSatDet_NumSamples_en_i  <= write_addr_valid;
      |                 elsif (unsigned(write_linear_addr_i) = 5) then
      |                     -- regSatDet_SaturationThreshold din/en
      |                     sm_regSatDet_SaturationThreshold_din_i <= S_AXI_WDATA;
      |                     sm_regSatDet_SaturationThreshold_en_i  <= write_addr_valid;
      |                 elsif (unsigned(write_linear_addr_i) = 6) then
      |                     -- regAGC_ExtPktDet_DelayCount din/en
      |                     sm_regAGC_ExtPktDet_DelayCount_din_i <= S_AXI_WDATA;
      |                     sm_regAGC_ExtPktDet_DelayCount_en_i  <= write_addr_valid;
      |                 elsif (unsigned(write_linear_addr_i) = 7) then
      |                     -- regAGC_targetRxInputPwr din/en
      |                     sm_regAGC_targetRxInputPwr_din_i <= S_AXI_WDATA;
      |                     sm_regAGC_targetRxInputPwr_en_i  <= write_addr_valid;
      |                 elsif (unsigned(write_linear_addr_i) = 8) then
      |                     -- regAGC_AutoCorr_MinPower din/en
      |                     sm_regAGC_AutoCorr_MinPower_din_i <= S_AXI_WDATA;
      |                     sm_regAGC_AutoCorr_MinPower_en_i  <= write_addr_valid;
      |                 elsif (unsigned(write_linear_addr_i) = 9) then
      |                     -- regAGC_AutoCorr_MinPktDuration din/en
      |                     sm_regAGC_AutoCorr_MinPktDuration_din_i <= S_AXI_WDATA;
      |                     sm_regAGC_AutoCorr_MinPktDuration_en_i  <= write_addr_valid;
      |                 elsif (unsigned(write_linear_addr_i) = 10) then
      |                     -- regAGC_WSDAGCCtrl din/en
      |                     sm_regAGC_WSDAGCCtrl_din_i <= S_AXI_WDATA;
      |                     sm_regAGC_WSDAGCCtrl_en_i  <= write_addr_valid;
      |                 elsif (unsigned(write_linear_addr_i) = 11) then
      |                     -- regAGC_AutoCorr_RatioThresh din/en
      |                     sm_regAGC_AutoCorr_RatioThresh_din_i <= S_AXI_WDATA;
      |                     sm_regAGC_AutoCorr_RatioThresh_en_i  <= write_addr_valid;
      |                 elsif (unsigned(write_linear_addr_i) = 12) then
      |                     -- regAGC_ManualRxVGA1_Gain din/en
      |                     sm_regAGC_ManualRxVGA1_Gain_din_i <= S_AXI_WDATA;
      |                     sm_regAGC_ManualRxVGA1_Gain_en_i  <= write_addr_valid;
      |                 elsif (unsigned(write_linear_addr_i) = 13) then
      |                     -- regAGC_ManualRxLNA_Gain din/en
      |                     sm_regAGC_ManualRxLNA_Gain_din_i <= S_AXI_WDATA;
      |                     sm_regAGC_ManualRxLNA_Gain_en_i  <= write_addr_valid;
      |                 elsif (unsigned(write_linear_addr_i) = 14) then
      |                     -- regAGC_ManualRxVGA2_Gain din/en
      |                     sm_regAGC_ManualRxVGA2_Gain_din_i <= S_AXI_WDATA;
      |                     sm_regAGC_ManualRxVGA2_Gain_en_i  <= write_addr_valid;
      |                 elsif (unsigned(write_linear_addr_i) = 15) then
      |                     -- regAGC_AutoCorr_LagTime din/en
      |                     sm_regAGC_AutoCorr_LagTime_din_i <= S_AXI_WDATA;
      |                     sm_regAGC_AutoCorr_LagTime_en_i  <= write_addr_valid;
      |                 elsif (unsigned(write_linear_addr_i) = 16) then
      |                     -- regAGC_pktDetPwr_absoluteThreshold_dBm din/en
      |                     sm_regAGC_pktDetPwr_absoluteThreshold_dBm_din_i <= S_AXI_WDATA;
      |                     sm_regAGC_pktDetPwr_absoluteThreshold_dBm_en_i  <= write_addr_valid;
      |                 elsif (unsigned(write_linear_addr_i) = 17) then
      |                     -- regAGC_pktDetPwr_detectLag din/en
      |                     sm_regAGC_pktDetPwr_detectLag_din_i <= S_AXI_WDATA;
      |                     sm_regAGC_pktDetPwr_detectLag_en_i  <= write_addr_valid;
      |                 elsif (unsigned(write_linear_addr_i) = 18) then
      |                     -- regAGC_NumFineGainSteps din/en
      |                     sm_regAGC_NumFineGainSteps_din_i <= S_AXI_WDATA;
      |                     sm_regAGC_NumFineGainSteps_en_i  <= write_addr_valid;
      |                 elsif (unsigned(write_linear_addr_i) = 19) then
      |                     -- regAGC_WSD_CCAThreshold_dBm din/en
      |                     sm_regAGC_WSD_CCAThreshold_dBm_din_i <= S_AXI_WDATA;
      |                     sm_regAGC_WSD_CCAThreshold_dBm_en_i  <= write_addr_valid;
      |                 elsif (unsigned(write_linear_addr_i) = 20) then
      |                     -- regAGC_LongCorr_Threshold din/en
      |                     sm_regAGC_LongCorr_Threshold_din_i <= S_AXI_WDATA;
      |                     sm_regAGC_LongCorr_Threshold_en_i  <= write_addr_valid;
      |                 elsif (unsigned(write_linear_addr_i) = 21) then
      |                     -- regAGC_pktDetPwr_deltaThreshold_dBm din/en
      |                     sm_regAGC_pktDetPwr_deltaThreshold_dBm_din_i <= S_AXI_WDATA;
      |                     sm_regAGC_pktDetPwr_deltaThreshold_dBm_en_i  <= write_addr_valid;
      |                 elsif (unsigned(write_linear_addr_i) = 22) then
      |                     -- regAGC_SPITIMINGFUDGE din/en
      |                     sm_regAGC_SPITIMINGFUDGE_din_i <= S_AXI_WDATA;
      |                     sm_regAGC_SPITIMINGFUDGE_en_i  <= write_addr_valid;
      |                 end if;
      |             end if;        
      |         
      |         
      |         end if;
      |     end if;
      | end process Write_Linear_Addr_Decode;
      |  
      | -----------------------------------------------------------------------------
      | -- READ Control
      | -----------------------------------------------------------------------------
      | 
      | S_AXI_RDATA  <= S_AXI_RDATA_i;
      | S_AXI_RVALID  <= S_AXI_RVALID_i;
      | S_AXI_RLAST   <= S_AXI_RLAST_i;
      | S_AXI_RID     <= S_AXI_RID_i;
      | -- TODO: no error checking
      | S_AXI_RRESP <= (others=>'0');
      | 
      | PROC_ARREADY_ACK: process(read_state, S_AXI_ARVALID, write_state, S_AXI_AWVALID) is begin
      |     -- Note: WRITE has higher priority than READ
      |     if (read_state = IDLE and S_AXI_ARVALID = '1' and write_state = IDLE and S_AXI_AWVALID /= '1') then
      |         S_AXI_ARREADY <= S_AXI_ARVALID;
      |     else
      |         S_AXI_ARREADY <= '0';
      |     end if;
      | end process PROC_ARREADY_ACK;
      | 
      | S_AXI_WREADY_i <= write_ready;
      | 
      | Process_Sideband: process(write_state, read_state) is begin
      |     if (read_state = READ_PREP) then
      |         s_shram_en <= '1';
      |     elsif (read_state = READ_DATA) then
      |         s_shram_en <= S_AXI_RREADY;
      |     elsif (write_state = WRITE_DATA) then
      |         s_shram_en <= S_AXI_WVALID;
      |     else
      |         s_shram_en <= '0';
      |     end if;
      | end process Process_Sideband;
      | 
      | Cmd_Decode_Read: process(AXI_AClk) is begin
      |     if (AXI_AClk'event and AXI_AClk = '1') then
      |         if (AXI_AResetN = '0') then
      |             S_AXI_RVALID_i <= '0';
      |             read_bank_addr_i    <= (others => '0');
      |             read_linear_addr_i  <= (others => '0');
      |             S_AXI_ARLEN_i       <= (others => '0');
      |             S_AXI_RLAST_i       <= '0';
      |             S_AXI_RID_i         <= (others => '0');
      |             read_state          <= IDLE;
      |             read_prep_counter   <= (others => '0');
      |             read_addr_counter   <= (others => '0');
      |             read_data_counter   <= (others => '0');
      |         else
      |             -- default assignments
      |             s_fifo_re <= '0';
      | 
      |             if (read_state = IDLE) then
      |                 -- Note WRITE has higher priority than READ
      |                 if (S_AXI_ARVALID = '1' and write_state = IDLE and S_AXI_AWVALID /= '1') then
      |                     -- extract bank and linear addresses
      |                     read_bank_addr_i    <= S_AXI_ARADDR(C_S_AXI_TOTAL_ADDR_LEN-1 downto C_S_AXI_LINEAR_ADDR_LEN+2);
      |                     read_linear_addr_i  <= S_AXI_ARADDR(C_S_AXI_LINEAR_ADDR_LEN+1 downto 2);
      |                     s_fifo_re <= '1';
      | 
      |                     -- reflect arid
      |                     S_AXI_RID_i <= S_AXI_ARID;
      | 
      |                     -- load read liner address and data counter
      |                     read_addr_counter <= S_AXI_ARLEN;
      |                     read_data_counter <= S_AXI_ARLEN;
      | 
      |                     -- load read preparation counter
      |                     read_prep_counter <= C_READ_PREP_DELAY;
      |                     -- read state transition
      |                     read_state <= READ_PREP;
      |                 end if;
      |             elsif (read_state = READ_PREP) then
      |                 if (unsigned(read_prep_counter) = 0) then
      |                     if (unsigned(read_data_counter) = 0) then
      |                         -- tag the last data generated by the slave
      |                         S_AXI_RLAST_i <= '1';
      |                     end if;
      |                     -- valid data appears
      |                     S_AXI_RVALID_i <= '1';
      |                     -- read state transition
      |                     read_state <= READ_DATA;
      |                 else
      |                     -- decrease read preparation counter
      |                     read_prep_counter <= Std_Logic_Vector(unsigned(read_prep_counter) - 1);
      |                 end if;
      | 
      |                 if (unsigned(read_prep_counter) /= 3 and unsigned(read_addr_counter) /= 0) then
      |                     -- decrease address counter
      |                     read_addr_counter <= Std_Logic_Vector(unsigned(read_addr_counter) - 1);
      |                     -- increase linear address (no band crossing)
      |                     read_linear_addr_i <= Std_Logic_Vector(unsigned(read_linear_addr_i) + 1);
      |                 end if;
      |             elsif (read_state = READ_DATA) then
      |                 if (S_AXI_RREADY = '1') then
      |                     if (unsigned(read_data_counter) = 1) then
      |                         -- tag the last data generated by the slave
      |                         S_AXI_RLAST_i <= '1';
      |                     end if;
      | 
      |                     if (unsigned(read_data_counter) = 0) then
      |                         -- arid
      |                         S_AXI_RID_i <= (others => '0');
      |                         -- rlast
      |                         S_AXI_RLAST_i <= '0';
      |                         -- no more valid data
      |                         S_AXI_RVALID_i <= '0';
      |                         -- read state transition
      |                         read_state <= IDLE;
      |                     else
      |                         -- decrease read preparation counter
      |                         read_data_counter <= Std_Logic_Vector(unsigned(read_data_counter) - 1);
      | 
      |                         if (unsigned(read_addr_counter) /= 0) then
      |                             -- decrease address counter
      |                             read_addr_counter <= Std_Logic_Vector(unsigned(read_addr_counter) - 1);
      |                             -- increase linear address (no band crossing)
      |                             read_linear_addr_i <= Std_Logic_Vector(unsigned(read_linear_addr_i) + 1);
      |                         end if;
      |                     end if;
      |                 end if;
      |             end if;
      | 
      |         end if;
      |     end if;
      | end process Cmd_Decode_Read;
      | 
      | Read_Linear_Addr_Decode : process(AXI_AClk) is begin
      |     if (AXI_AClk'event and AXI_AClk = '1') then
      |         if (AXI_AResetN = '0') then
      |             reg_bank_out_i   <= (others => '0');
      |             fifo_bank_out_i  <= (others => '0');
      |             shmem_bank_out_i <= (others => '0');
      |             S_AXI_RDATA_i    <= (others => '0');
      |         else
      |             if (unsigned(read_bank_addr_i) = 2) then
      |                 -- 'From Register'
      |                 if (unsigned(read_linear_addr_i) = 23) then
      |                     -- 'regSatDet_SaturationDetected' dout
      |                     reg_bank_out_i <= sm_regSatDet_SaturationDetected_dout_i;
      |                 elsif (unsigned(read_linear_addr_i) = 24) then
      |                     -- 'regWSD_RXGAIN_READ' dout
      |                     reg_bank_out_i <= sm_regWSD_RXGAIN_READ_dout_i;
      |                 elsif (unsigned(read_linear_addr_i) = 25) then
      |                     -- 'regWSD_RSSI' dout
      |                     reg_bank_out_i <= sm_regWSD_RSSI_dout_i;
      |                 elsif (unsigned(read_linear_addr_i) = 26) then
      |                     -- 'regWSD_meanPower' dout
      |                     reg_bank_out_i <= sm_regWSD_meanPower_dout_i;
      |                 elsif (unsigned(read_linear_addr_i) = 27) then
      |                     -- 'regWSD_MeanDC_Q' dout
      |                     reg_bank_out_i <= sm_regWSD_MeanDC_Q_dout_i;
      |                 elsif (unsigned(read_linear_addr_i) = 28) then
      |                     -- 'regWSD_MeanDC_I' dout
      |                     reg_bank_out_i <= sm_regWSD_MeanDC_I_dout_i;
      |                 elsif (unsigned(read_linear_addr_i) = 29) then
      |                     -- 'regWSD_RxLNAGain' dout
      |                     reg_bank_out_i <= sm_regWSD_RxLNAGain_dout_i;
      |                 elsif (unsigned(read_linear_addr_i) = 30) then
      |                     -- 'regWSD_RxVGA1Gain' dout
      |                     reg_bank_out_i <= sm_regWSD_RxVGA1Gain_dout_i;
      |                 elsif (unsigned(read_linear_addr_i) = 31) then
      |                     -- 'regWSD_RxVGA2Gain' dout
      |                     reg_bank_out_i <= sm_regWSD_RxVGA2Gain_dout_i;
      |                 end if;
      |                 -- 'To Register' (with register readback)
      |                 if (unsigned(read_linear_addr_i) = 0) then
      |                     -- 'regAGC_DefaultGainSettings' dout
      |                     reg_bank_out_i <= sm_regAGC_DefaultGainSettings_dout_i;
      |                 elsif (unsigned(read_linear_addr_i) = 1) then
      |                     -- 'regSPICtrl_SPIWriteDelay' dout
      |                     reg_bank_out_i <= sm_regSPICtrl_SPIWriteDelay_dout_i;
      |                 elsif (unsigned(read_linear_addr_i) = 2) then
      |                     -- 'regPwrMeas_AvgLength' dout
      |                     reg_bank_out_i <= sm_regPwrMeas_AvgLength_dout_i;
      |                 elsif (unsigned(read_linear_addr_i) = 3) then
      |                     -- 'regSatDet_SaturationMaxCount' dout
      |                     reg_bank_out_i <= sm_regSatDet_SaturationMaxCount_dout_i;
      |                 elsif (unsigned(read_linear_addr_i) = 4) then
      |                     -- 'regSatDet_NumSamples' dout
      |                     reg_bank_out_i <= sm_regSatDet_NumSamples_dout_i;
      |                 elsif (unsigned(read_linear_addr_i) = 5) then
      |                     -- 'regSatDet_SaturationThreshold' dout
      |                     reg_bank_out_i <= sm_regSatDet_SaturationThreshold_dout_i;
      |                 elsif (unsigned(read_linear_addr_i) = 6) then
      |                     -- 'regAGC_ExtPktDet_DelayCount' dout
      |                     reg_bank_out_i <= sm_regAGC_ExtPktDet_DelayCount_dout_i;
      |                 elsif (unsigned(read_linear_addr_i) = 7) then
      |                     -- 'regAGC_targetRxInputPwr' dout
      |                     reg_bank_out_i <= sm_regAGC_targetRxInputPwr_dout_i;
      |                 elsif (unsigned(read_linear_addr_i) = 8) then
      |                     -- 'regAGC_AutoCorr_MinPower' dout
      |                     reg_bank_out_i <= sm_regAGC_AutoCorr_MinPower_dout_i;
      |                 elsif (unsigned(read_linear_addr_i) = 9) then
      |                     -- 'regAGC_AutoCorr_MinPktDuration' dout
      |                     reg_bank_out_i <= sm_regAGC_AutoCorr_MinPktDuration_dout_i;
      |                 elsif (unsigned(read_linear_addr_i) = 10) then
      |                     -- 'regAGC_WSDAGCCtrl' dout
      |                     reg_bank_out_i <= sm_regAGC_WSDAGCCtrl_dout_i;
      |                 elsif (unsigned(read_linear_addr_i) = 11) then
      |                     -- 'regAGC_AutoCorr_RatioThresh' dout
      |                     reg_bank_out_i <= sm_regAGC_AutoCorr_RatioThresh_dout_i;
      |                 elsif (unsigned(read_linear_addr_i) = 12) then
      |                     -- 'regAGC_ManualRxVGA1_Gain' dout
      |                     reg_bank_out_i <= sm_regAGC_ManualRxVGA1_Gain_dout_i;
      |                 elsif (unsigned(read_linear_addr_i) = 13) then
      |                     -- 'regAGC_ManualRxLNA_Gain' dout
      |                     reg_bank_out_i <= sm_regAGC_ManualRxLNA_Gain_dout_i;
      |                 elsif (unsigned(read_linear_addr_i) = 14) then
      |                     -- 'regAGC_ManualRxVGA2_Gain' dout
      |                     reg_bank_out_i <= sm_regAGC_ManualRxVGA2_Gain_dout_i;
      |                 elsif (unsigned(read_linear_addr_i) = 15) then
      |                     -- 'regAGC_AutoCorr_LagTime' dout
      |                     reg_bank_out_i <= sm_regAGC_AutoCorr_LagTime_dout_i;
      |                 elsif (unsigned(read_linear_addr_i) = 16) then
      |                     -- 'regAGC_pktDetPwr_absoluteThreshold_dBm' dout
      |                     reg_bank_out_i <= sm_regAGC_pktDetPwr_absoluteThreshold_dBm_dout_i;
      |                 elsif (unsigned(read_linear_addr_i) = 17) then
      |                     -- 'regAGC_pktDetPwr_detectLag' dout
      |                     reg_bank_out_i <= sm_regAGC_pktDetPwr_detectLag_dout_i;
      |                 elsif (unsigned(read_linear_addr_i) = 18) then
      |                     -- 'regAGC_NumFineGainSteps' dout
      |                     reg_bank_out_i <= sm_regAGC_NumFineGainSteps_dout_i;
      |                 elsif (unsigned(read_linear_addr_i) = 19) then
      |                     -- 'regAGC_WSD_CCAThreshold_dBm' dout
      |                     reg_bank_out_i <= sm_regAGC_WSD_CCAThreshold_dBm_dout_i;
      |                 elsif (unsigned(read_linear_addr_i) = 20) then
      |                     -- 'regAGC_LongCorr_Threshold' dout
      |                     reg_bank_out_i <= sm_regAGC_LongCorr_Threshold_dout_i;
      |                 elsif (unsigned(read_linear_addr_i) = 21) then
      |                     -- 'regAGC_pktDetPwr_deltaThreshold_dBm' dout
      |                     reg_bank_out_i <= sm_regAGC_pktDetPwr_deltaThreshold_dBm_dout_i;
      |                 elsif (unsigned(read_linear_addr_i) = 22) then
      |                     -- 'regAGC_SPITIMINGFUDGE' dout
      |                     reg_bank_out_i <= sm_regAGC_SPITIMINGFUDGE_dout_i;
      |                 end if;
      | 
      |                 S_AXI_RDATA_i <= reg_bank_out_i;
      |             elsif (unsigned(read_bank_addr_i) = 1) then
      |                 -- 'From FIFO'
      |                 -- 'To FIFO'
      | 
      |                 S_AXI_RDATA_i <= fifo_bank_out_i;
      |             elsif (unsigned(read_bank_addr_i) = 0 and s_shram_en = '1') then
      |                 -- 'Shared Memory'
      | 
      |                 S_AXI_RDATA_i <= shmem_bank_out_i;
      |             end if;
      |         end if;
      |     end if;
      | end process Read_Linear_Addr_Decode;
      | 
      | end architecture IMP;
      settings: infoedit=For use with EDK Processor block.
  wires:
  memmap/23 -> To Register5/2
  memmap/22 -> To Register5/1
  memmap/19 -> To Register3/2
  memmap/18 -> To Register3/1
  memmap/21 -> To Register4/2
  memmap/20 -> To Register4/1
  memmap/15 -> To Register1/2
  memmap/14 -> To Register1/1
  memmap/17 -> To Register2/2
  memmap/16 -> To Register2/1
  memmap/27 -> To Register7/2
  memmap/26 -> To Register7/1
  memmap/47 -> To Register17/2
  memmap/46 -> To Register17/1
  memmap/55 -> To Register21/2
  memmap/54 -> To Register21/1
  memmap/45 -> To Register16/2
  memmap/44 -> To Register16/1
  memmap/51 -> To Register19/2
  memmap/50 -> To Register19/1
  memmap/33 -> To Register10/2
  memmap/32 -> To Register10/1
  memmap/57 -> To Register22/2
  memmap/56 -> To Register22/1
  memmap/49 -> To Register18/2
  memmap/48 -> To Register18/1
  memmap/41 -> To Register14/2
  memmap/40 -> To Register14/1
  memmap/37 -> To Register12/2
  memmap/36 -> To Register12/1
  memmap/39 -> To Register13/2
  memmap/38 -> To Register13/1
  memmap/53 -> To Register20/2
  memmap/52 -> To Register20/1
  memmap/25 -> To Register6/2
  memmap/24 -> To Register6/1
  memmap/13 -> To Register/2
  memmap/12 -> To Register/1
  memmap/35 -> To Register11/2
  memmap/34 -> To Register11/1
  memmap/29 -> To Register8/2
  memmap/28 -> To Register8/1
  memmap/31 -> To Register9/2
  memmap/30 -> To Register9/1
  memmap/43 -> To Register15/2
  memmap/42 -> To Register15/1
  memmap/11 -> S_AXI_WREADY/1
  memmap/10 -> S_AXI_RVALID/1
  memmap/9 -> S_AXI_RRESP/1
  memmap/8 -> S_AXI_RLAST/1
  memmap/7 -> S_AXI_RID/1
  memmap/6 -> S_AXI_RDATA/1
  memmap/5 -> S_AXI_BVALID/1
  memmap/4 -> S_AXI_BRESP/1
  memmap/3 -> S_AXI_BID/1
  memmap/2 -> S_AXI_AWREADY/1
  memmap/1 -> S_AXI_ARREADY/1
  S_AXI_WVALID/1 -> memmap/25
  S_AXI_WSTRB/1 -> memmap/24
  S_AXI_WLAST/1 -> memmap/23
  S_AXI_WDATA/1 -> memmap/22
  S_AXI_RREADY/1 -> memmap/21
  S_AXI_BREADY/1 -> memmap/20
  S_AXI_AWVALID/1 -> memmap/19
  S_AXI_AWSIZE/1 -> memmap/18
  S_AXI_AWPROT/1 -> memmap/17
  S_AXI_AWLOCK/1 -> memmap/16
  S_AXI_AWLEN/1 -> memmap/15
  S_AXI_AWID/1 -> memmap/14
  S_AXI_AWCACHE/1 -> memmap/13
  S_AXI_AWBURST/1 -> memmap/12
  S_AXI_AWADDR/1 -> memmap/11
  S_AXI_ARVALID/1 -> memmap/10
  S_AXI_ARSIZE/1 -> memmap/9
  S_AXI_ARPROT/1 -> memmap/8
  S_AXI_ARLOCK/1 -> memmap/7
  S_AXI_ARLEN/1 -> memmap/6
  S_AXI_ARID/1 -> memmap/5
  S_AXI_ARCACHE/1 -> memmap/4
  S_AXI_ARBURST/1 -> memmap/3
  S_AXI_ARADDR/1 -> memmap/2
  AXI_ARESETN/1 -> memmap/1
  From Register3/1 -> memmap/29
  From Register8/1 -> memmap/34
  From Register7/1 -> memmap/33
  From Register6/1 -> memmap/32
  From Register1/1 -> memmap/27
  From Register2/1 -> memmap/28
  From Register4/1 -> memmap/30
  From Register5/1 -> memmap/31
  To Register5/1 -> memmap/40
  To Register3/1 -> memmap/38
  From Register/1 -> memmap/26
  To Register4/1 -> memmap/39
  To Register1/1 -> memmap/36
  To Register2/1 -> memmap/37
  To Register7/1 -> memmap/42
  To Register17/1 -> memmap/52
  To Register21/1 -> memmap/56
  To Register16/1 -> memmap/51
  To Register19/1 -> memmap/54
  To Register10/1 -> memmap/45
  To Register22/1 -> memmap/57
  To Register18/1 -> memmap/53
  To Register14/1 -> memmap/49
  To Register12/1 -> memmap/47
  To Register13/1 -> memmap/48
  To Register20/1 -> memmap/55
  To Register6/1 -> memmap/41
  To Register/1 -> memmap/35
  To Register11/1 -> memmap/46
  To Register8/1 -> memmap/43
  To Register9/1 -> memmap/44
  To Register15/1 -> memmap/50
  S_AXI_WREADY/1 -> Terminator10/1
  S_AXI_RVALID/1 -> Terminator9/1
  S_AXI_RRESP/1 -> Terminator8/1
  S_AXI_RLAST/1 -> Terminator7/1
  S_AXI_RID/1 -> Terminator6/1
  S_AXI_RDATA/1 -> Terminator5/1
  S_AXI_BVALID/1 -> Terminator4/1
  S_AXI_BRESP/1 -> Terminator3/1
  S_AXI_BID/1 -> Terminator2/1
  S_AXI_AWREADY/1 -> Terminator1/1
  S_AXI_ARREADY/1 -> Terminator/1
  Constant24/1 -> S_AXI_WVALID/1
  Constant23/1 -> S_AXI_WSTRB/1
  Constant22/1 -> S_AXI_WLAST/1
  Constant21/1 -> S_AXI_WDATA/1
  Constant20/1 -> S_AXI_RREADY/1
  Constant19/1 -> S_AXI_BREADY/1
  Constant18/1 -> S_AXI_AWVALID/1
  Constant17/1 -> S_AXI_AWSIZE/1
  Constant16/1 -> S_AXI_AWPROT/1
  Constant15/1 -> S_AXI_AWLOCK/1
  Constant14/1 -> S_AXI_AWLEN/1
  Constant13/1 -> S_AXI_AWID/1
  Constant12/1 -> S_AXI_AWCACHE/1
  Constant11/1 -> S_AXI_AWBURST/1
  Constant10/1 -> S_AXI_AWADDR/1
  Constant9/1 -> S_AXI_ARVALID/1
  Constant8/1 -> S_AXI_ARSIZE/1
  Constant7/1 -> S_AXI_ARPROT/1
  Constant6/1 -> S_AXI_ARLOCK/1
  Constant5/1 -> S_AXI_ARLEN/1
  Constant4/1 -> S_AXI_ARID/1
  Constant3/1 -> S_AXI_ARCACHE/1
  Constant2/1 -> S_AXI_ARBURST/1
  Constant1/1 -> S_AXI_ARADDR/1
  Constant/1 -> AXI_ARESETN/1
